simulink model "TestbedModel_v6"  (R2016a)
settings: Solver=ode23tb  StartTime=0.0  StopTime=20  RelTol=1e-3
undefined symbols (not defined in the file): K, Ki, Kp, magnitude, rev_comms_sink, tau
libraries: DAEMOT_Lib x4
(part 1 of 4)
settings Model: Creator=aksland2  LastModifiedBy=aksland2

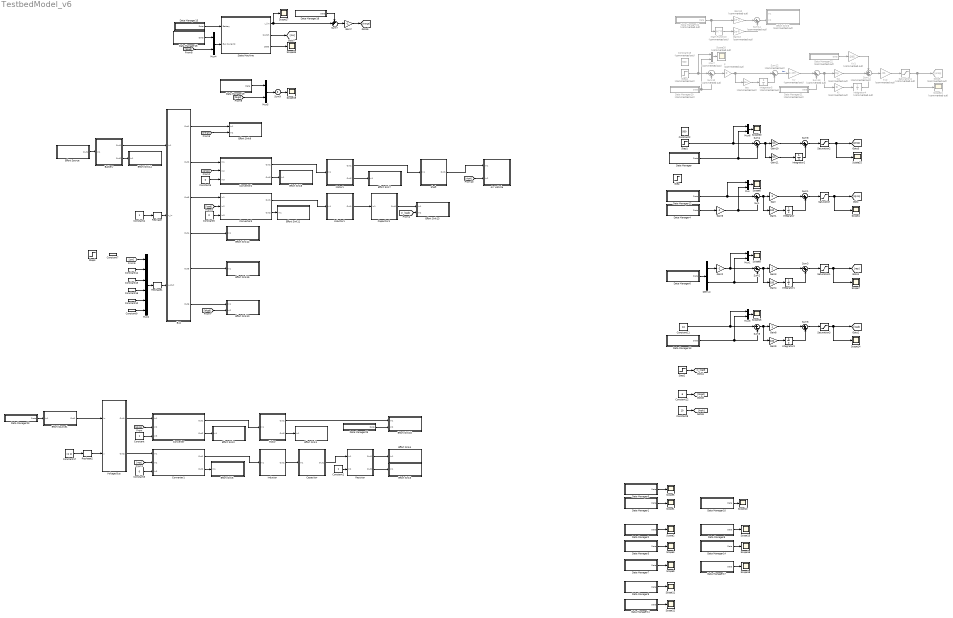
== system TestbedModel_v6 ==
  Air Vehicle : Subsystem  AncestorBlock=DAEMOT_Lib/Dyn Electrical Comp/Air Vehicle  mask{rho=1.225, g=9.81, M=69.5*.4536, A=2*pi*.3^2, C_D=1.5/45, v_initial=0, prop=AFRL}
      mask prompts: rho "Air Density [kg/m^3]"; g "Gravity [m/s^2]"; M "Vehicle Mass [kg]"; A "Frontal Area [m^2]"; C_D "Drag Coefficient [-]"; v_initial "Initial Vehicle Speed [m/s]"; prop "Propeller Map (filename)"
      mask init:
      | map = load('PropellerProp','PropellerProp');
      | Prop = eval(['map.PropellerProp.' prop]);
      | d = Prop.d;
      settings: CopyFcn=|
      | h      = get_param(gcb,'handle');   % Get block handle
      | blk    = gcb;
      | 
      | set_param(blk, 'LinkStatus', 'inactive')
      | clear h
      | clear blk
      mask Display:
      | image(imread('UAV.bmp'));
      | text(0.5,0.95,['{\bf UAV}'],'TexMode','on','horizontalAlignment', 'center')
      | text(0.5,0.075,['{\bf (\tau)  (end)}'],'TexMode','on','horizontalAlignment', 'center')
      | 
      | port_label('input',1,sprintf('Mechanical \nIn'))
      | % port_label('input',2,sprintf('\\lambda %g\t',10))
      | port_label('input',2,'\theta [rad]','interpreter','tex')
  Battery : Subsystem  AncestorBlock=DAEMOT_Lib/Dyn Electrical Comp/Battery  mask{C_c=62.7, C_s=4.5, R_cond=1.94, B_cap=21.33, Ns=1, Np=1, batt=57.6 Testbed 21.33 Ah, Ts_initial=25, Tc_initial=25, SOC_initial=.75, RC_initial=[0 0]}
      mask prompts: C_c "Lumped Cell Core Heat Capacity [J/K]"; C_s "Lumped Cell Surface Heat Capacity [J/K]"; R_cond "Conduction Resistance  [K/W]"; B_cap "Battery Capacity [Ah]"; Ns "Number of Cells (Series)"; Np "Number of Cells (Parallel)"; batt "Battery Type"; Ts_initial "Initial Battery Surface Temperature [C]"; Tc_initial "Initial Battery Core Temperature [C]"; SOC_initial "Initial State of Charge"; RC_initial "Initial RC Pair Voltage"
      mask init:
      | load('BattProp.mat');
      | 
      | if strcmp(batt,'3.3V LiFePO4 2.3 Ah')
      |     cell = BattProp.LiFePO_33V;
      |     t = 1;
      | end
      | 
      | if strcmp(batt,'3.3V LiFePO4 Graph 2.3 Ah')
      |     cell = BattProp.LiFePO_33V_G;
      |     t = 2;
      | end
      | 
      | if strcmp(batt,'4.2V LiPo 5.1 Ah')
      |     cell = BattProp.LiPo_42V;
      |     t = 1;
      | end
      | 
      | if strcmp(batt,'4.2V LiPo Graph 5.1 Ah')
      |     cell = BattProp.LiPo_42V_G;
      |     t = 2;
      | end
      | 
      | if strcmp(batt,'57.6 Testbed 21.33 Ah')
      |     cell = BattProp.Testbed4Pack;
      |     t = 1;
      | end
      | 
      | if strcmp(batt,'57.6 Testbed Graph 21.33 Ah')
      |     cell = BattProp.Testbed4Pack_G;
      |     t = 2;
      | end
      | 
      | 
      | % B_cap = B_cap*Np;
      | % C_c = C_c*Np*Ns;
      | % C_s = C_s*Np*Ns;
      | % R_cond = R_cond/(Np*Ns);
      settings: CopyFcn=|
      | h      = get_param(gcb,'handle');   % Get block handle
      | blk    = gcb;
      | 
      | set_param(blk, 'LinkStatus', 'inactive')
      | clear h
      | clear blk
      mask TypeOptions batt: 3.3V LiFePO4 2.3 Ah | 3.3V LiFePO4 Graph 2.3 Ah | 4.2V LiPo 5.1 Ah | 4.2V LiPo Graph 5.1 Ah | 57.6 Testbed 21.33 Ah | 57.6 Testbed Graph 21.33 Ah
      mask Display:
      | image(imread('battery.bmp'))
      | N = get_param(gcb,'Np');
      | M = get_param(gcb,'Ns');
      | 
      | text(0.5,0.95,[M '{\bfS}' N '{\bfP Battery}'],'TexMode','on','horizontalAlignment', 'center')
      | text(0.5,0.075,['{\bf (V)*}'],'TexMode','on','horizontalAlignment', 'center')
      | 
      | port_label('input',1,sprintf('Electrical \nIn'))
      | 
      | port_label('output',1,sprintf('Electrical \nOut'))
      | port_label('output',2,sprintf('Cooling \nOut'))
  Bus : Subsystem  AncestorBlock=DAEMOT_Lib/Dyn Electrical Comp/Bus  mask{R=5e-4, L=4e-8, C=.01, Num_In=1, Num_Out=6, V_initial=60, I_initial=0}
      mask prompts: R "Resistance [Ohm]"; L "Inductance [H]"; C "Capacitance [F]"; Num_In "Number of Inputs"; Num_Out "Number of Outputs"; V_initial "Initial Voltage [V]"; I_initial "Initial Current [A]"
      mask init:
      | h      = get_param(gcb,'handle');   % Get block handle
      | blk    = gcb;
      | hblock = get(h);     % Parse out handles structure
      | 
      | %%%%%%%%%%%%%%%%%%%%%%%%%%%%%% Clear Stuff %%%%%%%%%%%%%%%%%%%%%%%%%%%%%%%%
      | %delete any previous inports and bus selectors
      | for i = str2num(hblock.Num_In)+1:hblock.Ports(1)-2
      |     delete_block([blk,'/In',num2str(i)])
      |     delete_block([blk,'/gb',num2str(i)])
      |     delete_block([blk,'/vm',num2str(i)])
      |     delete_block([blk,'/term',num2str(i)])
      |     delete_block([blk,'/Sink',num2str(i)])
      |     delete_block([blk,'/vin',num2str(i)])
      |     
      |     delete_unconnected_lines(blk)
      | end
      | 
      | for i = str2num(hblock.Num_Out)+1:hblock.Ports(2)
      |     delete_block([blk,'/Out',num2str(i)])
      |     delete_block([blk,'/if',num2str(i)])
      |     delete_block([blk,'/io',num2str(i)])
      |     delete_block([blk,'/vo',num2str(i)])
      |     delete_block([blk,'/vot',num2str(i)])
      |     delete_block([blk,'/b',num2str(i)])
      |     delete_block([blk,'/Source',num2str(i)])
      |     delete_block([blk,'/ig',num2str(i)])
      | %     delete_block([blk,'/ios',num2str(i)])
      |     
      |     delete_unconnected_lines(blk)
      | end
      | %%%%%%%%%%%%%%%%%%%%%%%%%%%%% Clear Stuff %%%%%%%%%%%%%%%%%%%%%%%%%%%%%%%%
      | 
      | %%%%%%%%%%%%%%%%%%%%%%%%%%%%%% Edit Mux inputs %%%%%%%%%%%%%%%%%%%%%%%%%%%%%%%%
      | set_param([blk,'/Mux_In_1'],'Inputs',hblock.Num_In)
      | set_param([blk,'/Mux_In_2'],'Inputs',hblock.Num_Out)
      | set_param([blk,'/Demux_Out_1'],'Outputs',hblock.Num_In)
      | set_param([blk,'/Demux_Out_2'],'Outputs',hblock.Num_Out)
      | set_param([blk,'/u_Out'],'Port',num2str(Num_In+2))
      | set_param([blk,'/u_In'],'Port',num2str(Num_In+1))
      | set_param([blk,'/Bus_Sink_1'],'Inputs',num2str(str2num(hblock.Num_In)+1))
      | set_param([blk,'/Demux_Out_3'],'Outputs',hblock.Num_In)
      | delete_unconnected_lines(blk)
      | 
      | %%%%%%%%%%%%%%%%%%%%%%%%%%%%%% Edit Mux inputs %%%%%%%%%%%%%%%%%%%%%%%%%%%%%%%%
      | 
      | %%%%%%%%%%%%%%%%%%%%%%%%%%%%%% Create and Place Inputs %%%%%%%%%%%%%%%%%%%%%%%%%%%%%%%%
      | % generate inports, bus selectors, and route lines to each vector concat
      | for i = hblock.Ports(1)+1-2:str2num(hblock.Num_In)
      |     
      |     % add blocks (positioning notation [x i*s+y x+l i*s+h+y] x:(horiz. pos.), y:(vert. pos.), s:(spacing), l:(horiz. length), x:(vert. height)
      |     add_block('simulink/Ports & Subsystems/In1',   [blk,'/In',num2str(i)],    'Position',[355 i*80+425 355+30 i*80+13+425]);         % adding inport
      |     add_block([blk,'/gb1'],                        [blk,'/gb',num2str(i)],   'Position',[440 i*80+410 440+5 i*80+38+410]);         % adding inport
      |     add_block('simulink/Signal Routing/Goto',      [blk,'/vm',num2str(i)],    'Position',[500 i*80+450 500+80 i*80+14+450]);         % adding inport
      |     add_block('simulink/Sinks/Terminator',          [blk,'/term',num2str(i)],    'Position',[500 i*80+415 500+20 i*80+14+415]);         % adding inport
      |     add_block('DAEMOT_Lib/Support Functions/Sink',[blk,'/Sink',num2str(i)],'Position',[200 i*30+336 200+65 i*30+28+336]);         % adding inport
      |     add_block('simulink/Signal Routing/From',       [blk,'/vin',num2str(i)],     'Position',[-400 i*20+405 -400+80 i*20+18+405]);         % adding inport
      |     
      |     % set goto and from tags
      |     set_param([blk,'/vm',num2str(i)],'GotoTag',char(horzcat('V_in',num2str(i))))
      |     set_param([blk,'/vin',num2str(i)],'GotoTag',char(horzcat('V_in',num2str(i))))
      |     
      |     % set goto and from background colors
      | %    set_param([blk,'/gm',num2str(i)],'BackgroundColor','yellow')
      | %    set_param([blk,'/gt',num2str(i)],'BackgroundColor','yellow')
      | %    %set_param([blk,'/gp',num2str(i)],'BackgroundColor','yellow')
      | %    set_param([blk,'/min',num2str(i)],'BackgroundColor','yellow')
      | %    set_param([blk,'/tin',num2str(i)],'BackgroundColor','yellow')
      | %    set_param([blk,'/pout',num2str(i)],'BackgroundColor','cyan')
      |     
      |     % add lines
      |     add_line(blk,['In',num2str(i),'/1'], ['gb',num2str(i),'/1'],'AutoRouting','on')
      |     add_line(blk,['gb',num2str(i),'/2'],  ['vm',num2str(i),'/1'],'AutoRouting','on')
      |     add_line(blk,['gb',num2str(i),'/1'],  ['term',num2str(i),'/1'],'AutoRouting','on')
      |     add_line(blk,['Demux_Out_1/',num2str(i)],  ['Sink',num2str(i),'/1'],'AutoRouting','on')
      |     add_line(blk,['vin',num2str(i),'/1'],  ['Mux_In_1/',num2str(i)],'AutoRouting','on')
      |     add_line(blk,['Demux_Out_3/',num2str(i)'],  ['Bus_Sink_1/',num2str(i)+1],'AutoRouting','on')
      |     
      |     p = get_param([blk,'/Demux_Out_3'],'PortHandles');
      |     l = get_param(p.Outport(i),'Line');
      |     set_param(l,'Name',['Current',num2str(i),' [A]'])
      | %     
      | end
      | %%%%%%%%%%%%%%%%%%%%%%%%%%%%%% Create and Place Inputs %%%%%%%%%%%%%%%%%%%%%%%%%%%%%%%%
      | 
      | %%%%%%%%%%%%%%%%%%%%%%%%%%%%%% Create and Place Outputs %%%%%%%%%%%%%%%%%%%%%%%%%%%%%%%%
      | % generate inports, bus selectors, and route lines to each vector concat
      | for i = hblock.Ports(2)+1:str2num(hblock.Num_Out)
      |     
      |     % add blocks
      |     add_block('simulink/Ports & Subsystems/Out1',   [blk,'/Out',num2str(i)],   'Position',[875 i*80+425 875+30 i*80+13+425]);         % adding inport
      |     add_block('simulink/Signal Routing/Bus Creator',[blk,'/b',num2str(i)],     'Position',[825 i*80+410 825+5 i*80+38+410]);         % adding inport
      |     add_block('simulink/Signal Routing/From',       [blk,'/io',num2str(i)],     'Position',[710 i*80+415 710+80 i*80+14+415]);         % adding inport
      |     add_block('simulink/Signal Routing/From',       [blk,'/vo',num2str(i)],     'Position',[710 i*80+435 710+80 i*80+14+435]);         % adding inport
      |     add_block('simulink/Signal Routing/Goto',       [blk,'/vot',num2str(i)],     'Position',[1250 i*20+50 1250+80 i*20+18+50]);         % adding inport
      |     add_block('simulink/Signal Routing/From',       [blk,'/if',num2str(i)],     'Position',[935 i*20+410 935+80 i*20+18+410]);         % adding inport
      |     add_block('DAEMOT_Lib/Support Functions/Source',[blk,'/Source',num2str(i)],'Position',[1400 i*30+420 1400+65 i*30+28+420]);         % adding inport
      |     add_block('simulink/Signal Routing/Goto',       [blk,'/ig',num2str(i)],     'Position',[1550 i*30+430 1550+80 i*30+14+430]);         % adding inport
      | %     add_block('simulink/Signal Routing/From',       [blk,'/ios',num2str(i)],     'Position',[1770 i*16+405 1770+80 i*16+14+405]);         % adding inport
      |     
      |     % set goto and from tags
      |     set_param([blk,'/if',num2str(i)],'GotoTag',char(horzcat('I_out',num2str(i))))
      |     set_param([blk,'/io',num2str(i)],'GotoTag',char(horzcat('I_out',num2str(i))))
      |     set_param([blk,'/vo',num2str(i)],'GotoTag',char(horzcat('V_out',num2str(i))))
      |     set_param([blk,'/vot',num2str(i)],'GotoTag',char(horzcat('V_out',num2str(i))))
      |     set_param([blk,'/ig',num2str(i)],'GotoTag',char(horzcat('I_out',num2str(i))))
      | %     set_param([blk,'/ios',num2str(i)],'GotoTag',char(horzcat('I_out',num2str(i))))
      |     set_param([blk,'/b',num2str(i)],'Inputs','2')
      |     
      | %     % set goto and from background colors
      | %     set_param([blk,'/t',num2str(i)],'BackgroundColor','cyan')
      | %     set_param([blk,'/m',num2str(i)],'BackgroundColor','cyan')
      | %     set_param([blk,'/p',num2str(i)],'BackgroundColor','cyan')
      | %     set_param([blk,'/g',num2str(i)],'BackgroundColor','cyan')
      | %     set_param([blk,'/mout',num2str(i)],'BackgroundColor','cyan')
      | %     %set_param([blk,'/tout',num2str(i)],'BackgroundColor','cyan')
      |     
      |     % add lines
      |     add_line(blk,['io',num2str(i),'/1'],['b',num2str(i),'/1'],'AutoRouting','on')
      |     p = get_param([blk,'/io',num2str(i)],'PortHandles');
      |     l = get_param(p.Outport,'Line');
      |     set_param(l,'Name','current')
      |     
      |     add_line(blk,['vo',num2str(i),'/1'],['b',num2str(i),'/2'],'AutoRouting','on')
      |     p = get_param([blk,'/vo',num2str(i)],'PortHandles');
      |     l = get_param(p.Outport,'Line');
      |     set_param(l,'Name','voltage')
      |         
      | %     add_line(blk,['ios',num2str(i),'/1'],['Bus_Sink_1/',num2str(i+1)],'AutoRouting','on')
      | %     p = get_param([blk,'/ios',num2str(i)],'PortHandles');
      | %     l = get_param(p.Outport,'Line');
      | %     set_param(l,'Name',['Current',num2str(i),' [A]'])
      |      
      |     add_line(blk,['b',num2str(i),'/1'],['Out',num2str(i),'/1'],'AutoRouting','on')
      |     add_line(blk,['Source',num2str(i),'/1'],['ig',num2str(i),'/1'],'AutoRouting','on')
      |     add_line(blk,['if',num2str(i),'/1'],  ['Mux_In_2/',num2str(i)],'AutoRouting','on')
      |     add_line(blk,['Demux_Out_2/',num2str(i)],['vot',num2str(i),'/1'],'AutoRouting','on')
      |     
      | 
      | 
      | end
      | %%%%%%%%%%%%%%%%%%%%%%%%%%%%%% Create and Place Outputs %%%%%%%%%%%%%%%%%%%%%%%%%%%%%%%%
      | 
      | try
      |     set_param([blk,'/Selector1'],'InputPortWidth',num2str(hblock.Num_In))
      |     
      |     selector_str = '[1 ';
      |     for i = 2:str2num(hblock.Num_In)
      |         selector_str = [selector_str,num2str(i),' '];
      |     end
      |     selector_str = [selector_str,']'];
      |     set_param([blk,'/Selector1'],'IndexParamArray',{selector_str})%num2cell(1:hblock.Num_In))
      | catch
      |     selector_str = '[1 ';
      |     for i = 2:str2num(hblock.Num_In)
      |         selector_str = [selector_str,num2str(i),' '];
      |     end
      |     selector_str = [selector_str,']'];
      |     set_param([blk,'/Selector1'],'IndexParamArray',{selector_str})%num2cell(1:hblock.Num_In))
      |     
      |     set_param([blk,'/Selector1'],'InputPortWidth',num2str(hblock.Num_In))
      | end 
      |     
      | try
      |     set_param([blk,'/Selector2'],'InputPortWidth',num2str(hblock.Num_Out))
      |     
      |     selector_str = '[1 ';
      |     for i = 2:str2num(hblock.Num_Out)
      |         selector_str = [selector_str,num2str(i),' '];
      |     end
      |     selector_str = [selector_str,']'];
      |     set_param([blk,'/Selector2'],'IndexParamArray',{selector_str})%num2cell(1:hblock.Num_Out))
      | catch
      |     selector_str = '[1 ';
      |     for i = 2:str2num(hblock.Num_Out)
      |         selector_str = [selector_str,num2str(i),' '];
      |     end
      |     selector_str = [selector_str,']'];
      |     set_param([blk,'/Selector2'],'IndexParamArray',{selector_str})%num2cell(1:hblock.Num_Out))
      |     
      |     set_param([blk,'/Selector2'],'InputPortWidth',num2str(hblock.Num_Out))
      | end 
      | 
      |     clear h blk hblock
      settings: CopyFcn=|
      | h      = get_param(gcb,'handle');   % Get block handle
      | blk    = gcb;
      | 
      | set_param(blk, 'LinkStatus', 'inactive')
      | clear h
      | clear blk
      mask Display:
      | text(0.5,0.95,['{\bf Bus}'],'TexMode','on','horizontalAlignment', 'center')
      | text(0.5,0.075,['{\bf ----(V)}'],'TexMode','on','horizontalAlignment', 'center')
      | 
      | In = get_param(gcb,'Num_In');
      | Out = get_param(gcb,'Num_Out');
      | 
      | for i = 1:str2num(In)
      |     port_label('input',i,sprintf(['Electrical \nIn ',num2str(i)]))
      | end
      | port_label('input',str2num(In)+1,'u In')
      | port_label('input',str2num(In)+2,'u Out')
      | 
      | for i = 1:str2num(Out)
      |     port_label('output',i,sprintf(['Electrical \nOut ',num2str(i)]))
      | end
  Capacitor : Subsystem  AncestorBlock=DAEMOT_Lib/Dyn Electrical Comp/Capacitor  mask{C=.003, V_initial=0}
      mask prompts: C "Capacitance [F]"; V_initial "Initial Ouput Voltage [V]"
      mask init:
      | % if strcmp(Gn_check,'off')
      | %     %is not ground node
      | %     Gn = 0;
      | %     %V_initial = V_initial_temp;
      | % else
      | %     %is ground node
      | %     Gn = 1;
      | %     %V_initial = 0;
      | % end
      settings: CopyFcn=|
      | h      = get_param(gcb,'handle');   % Get block handle
      | blk    = gcb;
      | 
      | set_param(blk, 'LinkStatus', 'inactive')
      | clear h
      | clear blk
      mask Display:
      | image(imread('capacitor.bmp'));
      | text(0.5,0.95,['{\bf Capacitor}'],'TexMode','on','horizontalAlignment', 'center')
      | text(0.5,0.075,['{\bf (V)}'],'TexMode','on','horizontalAlignment', 'center')
      | 
      | port_label('input',1,sprintf('Electrical \nIn'))
      | %port_label('input',2,'Capacitance')
      | port_label('output',1,sprintf('Electrical \nOut'))
  Capacitor1 : Subsystem  AncestorBlock=DAEMOT_Lib/Dyn Electrical Comp/Capacitor  mask{C=.003, V_initial=24}
      mask prompts: C "Capacitance [F]"; V_initial "Initial Ouput Voltage [V]"
      mask init:
      | % if strcmp(Gn_check,'off')
      | %     %is not ground node
      | %     Gn = 0;
      | %     %V_initial = V_initial_temp;
      | % else
      | %     %is ground node
      | %     Gn = 1;
      | %     %V_initial = 0;
      | % end
      settings: CopyFcn=|
      | h      = get_param(gcb,'handle');   % Get block handle
      | blk    = gcb;
      | 
      | set_param(blk, 'LinkStatus', 'inactive')
      | clear h
      | clear blk
      mask Display:
      | image(imread('capacitor.bmp'));
      | text(0.5,0.95,['{\bf Capacitor}'],'TexMode','on','horizontalAlignment', 'center')
      | text(0.5,0.075,['{\bf (V)}'],'TexMode','on','horizontalAlignment', 'center')
      | 
      | port_label('input',1,sprintf('Electrical \nIn'))
      | %port_label('input',2,'Capacitance')
      | port_label('output',1,sprintf('Electrical \nOut'))
  Constant{,1,4,9..10,14..16} (8 alike) : Constant
  Constant11 : Constant  Value=24
  Constant12 : Constant  Value=.5
  Constant13 : Constant  Commented=on  Value=500
  Constant17 : Constant  Value=[1 1]
  Constant2 : Constant  Value=500
  Constant{3,5..7} (4 alike) : Constant  Value=0
  Constant8 : Constant  Value=10
  Converter : Subsystem  AncestorBlock=DAEMOT_Lib/Dyn Electrical Comp/Converter  mask{V_D=.01, R_D=.01, R_s=.01, R_L=.01, dir=<===, Cp=60, T_initial=25}
      mask prompts: V_D "Diode Voltage Difference [V]"; R_D "Diode Resistance [Ohm]"; R_s "Switch Resistance [Ohm]"; R_L "Copper Loss [Ohm]"; dir "Conversion Direction (Boost)"; Cp "Heat Capacity [J/K]"; T_initial "Initial Temperature [C]"
      settings: CopyFcn=|
      | h      = get_param(gcb,'handle');   % Get block handle
      | blk    = gcb;
      | 
      | set_param(blk, 'LinkStatus', 'inactive')
      | clear h
      | clear blk
      mask TypeOptions dir: ===> | <===
      mask Display:
      | image(imread('converter.bmp'));
      | text(0.5,0.95,['{\bf BuckBoost Converter}'],'TexMode','on','horizontalAlignment', 'center')
      | text(0.5,0.075,['{\bf ----(V)}'],'TexMode','on','horizontalAlignment', 'center')
      | dir = get_param(gcb,'dir');
      | 
      | switch dir
      |     case '===>'
      |         text(0.5,0.85,['{\bf Boost[1] ===>}'],'TexMode','on','horizontalAlignment', 'center')
      |         text(0.5,0.75,['{\bf Buck[0] <===}'],'TexMode','on','horizontalAlignment', 'center')
      |     case '<==='
      |         text(0.5,0.85,['{\bf Boost[1] <===}'],'TexMode','on','horizontalAlignment', 'center')
      |         text(0.5,0.75,['{\bf Buck[0] ===>}'],'TexMode','on','horizontalAlignment', 'center')
      | end
      | 
      | 
      | 
      | port_label('input',1,sprintf('Electrical \nIn'))
      | port_label('input',2,sprintf('Duty \nCycle'))
      | port_label('input',3,sprintf('Operating \nMode'))
      | port_label('output',1,sprintf('Electrical \nOut'))
      | port_label('output',2,sprintf('Cooling \nOut'))
  Converter1 : Subsystem  AncestorBlock=DAEMOT_Lib/Dyn Electrical Comp/Converter  mask{V_D=.01, R_D=.01, R_s=.01, R_L=.01, dir=<===, Cp=60, T_initial=25}
      mask prompts: V_D "Diode Voltage Difference [V]"; R_D "Diode Resistance [Ohm]"; R_s "Switch Resistance [Ohm]"; R_L "Copper Loss [Ohm]"; dir "Conversion Direction (Boost)"; Cp "Heat Capacity [J/K]"; T_initial "Initial Temperature [C]"
      settings: CopyFcn=|
      | h      = get_param(gcb,'handle');   % Get block handle
      | blk    = gcb;
      | 
      | set_param(blk, 'LinkStatus', 'inactive')
      | clear h
      | clear blk
      mask TypeOptions dir: ===> | <===
      mask Display:
      | image(imread('converter.bmp'));
      | text(0.5,0.95,['{\bf BuckBoost Converter}'],'TexMode','on','horizontalAlignment', 'center')
      | text(0.5,0.075,['{\bf ----(V)}'],'TexMode','on','horizontalAlignment', 'center')
      | dir = get_param(gcb,'dir');
      | 
      | switch dir
      |     case '===>'
      |         text(0.5,0.85,['{\bf Boost[1] ===>}'],'TexMode','on','horizontalAlignment', 'center')
      |         text(0.5,0.75,['{\bf Buck[0] <===}'],'TexMode','on','horizontalAlignment', 'center')
      |     case '<==='
      |         text(0.5,0.85,['{\bf Boost[1] <===}'],'TexMode','on','horizontalAlignment', 'center')
      |         text(0.5,0.75,['{\bf Buck[0] ===>}'],'TexMode','on','horizontalAlignment', 'center')
      | end
      | 
      | 
      | 
      | port_label('input',1,sprintf('Electrical \nIn'))
      | port_label('input',2,sprintf('Duty \nCycle'))
      | port_label('input',3,sprintf('Operating \nMode'))
      | port_label('output',1,sprintf('Electrical \nOut'))
      | port_label('output',2,sprintf('Cooling \nOut'))
  Converter2 : Subsystem  AncestorBlock=DAEMOT_Lib/Dyn Electrical Comp/Converter  mask{V_D=.05, R_D=.01, R_s=.01, R_L=.01, dir=<===, Cp=60, T_initial=25}
      mask prompts: V_D "Diode Voltage Difference [V]"; R_D "Diode Resistance [Ohm]"; R_s "Switch Resistance [Ohm]"; R_L "Copper Loss [Ohm]"; dir "Conversion Direction (Boost)"; Cp "Heat Capacity [J/K]"; T_initial "Initial Temperature [C]"
      settings: CopyFcn=|
      | h      = get_param(gcb,'handle');   % Get block handle
      | blk    = gcb;
      | 
      | set_param(blk, 'LinkStatus', 'inactive')
      | clear h
      | clear blk
      mask TypeOptions dir: ===> | <===
      mask Display:
      | image(imread('converter.bmp'));
      | text(0.5,0.95,['{\bf BuckBoost Converter}'],'TexMode','on','horizontalAlignment', 'center')
      | text(0.5,0.075,['{\bf ----(V)}'],'TexMode','on','horizontalAlignment', 'center')
      | dir = get_param(gcb,'dir');
      | 
      | switch dir
      |     case '===>'
      |         text(0.5,0.85,['{\bf Boost[1] ===>}'],'TexMode','on','horizontalAlignment', 'center')
      |         text(0.5,0.75,['{\bf Buck[0] <===}'],'TexMode','on','horizontalAlignment', 'center')
      |     case '<==='
      |         text(0.5,0.85,['{\bf Boost[1] <===}'],'TexMode','on','horizontalAlignment', 'center')
      |         text(0.5,0.75,['{\bf Buck[0] ===>}'],'TexMode','on','horizontalAlignment', 'center')
      | end
      | 
      | 
      | 
      | port_label('input',1,sprintf('Electrical \nIn'))
      | port_label('input',2,sprintf('Duty \nCycle'))
      | port_label('input',3,sprintf('Operating \nMode'))
      | port_label('output',1,sprintf('Electrical \nOut'))
      | port_label('output',2,sprintf('Cooling \nOut'))
  Converter3 : Subsystem  AncestorBlock=DAEMOT_Lib/Dyn Electrical Comp/Converter  mask{V_D=.05, R_D=.01, R_s=.01, R_L=.01, dir=<===, Cp=60, T_initial=25}
      mask prompts: V_D "Diode Voltage Difference [V]"; R_D "Diode Resistance [Ohm]"; R_s "Switch Resistance [Ohm]"; R_L "Copper Loss [Ohm]"; dir "Conversion Direction (Boost)"; Cp "Heat Capacity [J/K]"; T_initial "Initial Temperature [C]"
      settings: CopyFcn=|
      | h      = get_param(gcb,'handle');   % Get block handle
      | blk    = gcb;
      | 
      | set_param(blk, 'LinkStatus', 'inactive')
      | clear h
      | clear blk
      mask TypeOptions dir: ===> | <===
      mask Display:
      | image(imread('converter.bmp'));
      | text(0.5,0.95,['{\bf BuckBoost Converter}'],'TexMode','on','horizontalAlignment', 'center')
      | text(0.5,0.075,['{\bf ----(V)}'],'TexMode','on','horizontalAlignment', 'center')
      | dir = get_param(gcb,'dir');
      | 
      | switch dir
      |     case '===>'
      |         text(0.5,0.85,['{\bf Boost[1] ===>}'],'TexMode','on','horizontalAlignment', 'center')
      |         text(0.5,0.75,['{\bf Buck[0] <===}'],'TexMode','on','horizontalAlignment', 'center')
      |     case '<==='
      |         text(0.5,0.85,['{\bf Boost[1] <===}'],'TexMode','on','horizontalAlignment', 'center')
      |         text(0.5,0.75,['{\bf Buck[0] ===>}'],'TexMode','on','horizontalAlignment', 'center')
      | end
      | 
      | 
      | 
      | port_label('input',1,sprintf('Electrical \nIn'))
      | port_label('input',2,sprintf('Duty \nCycle'))
      | port_label('input',3,sprintf('Operating \nMode'))
      | port_label('output',1,sprintf('Electrical \nOut'))
      | port_label('output',2,sprintf('Cooling \nOut'))
  Data Manager : Subsystem  AncestorBlock=DAEMOT_Lib/Support Functions/Data Manager  mask{null=0}
      mask init:
      | set_param(gcb, 'LinkStatus', 'inactive')    % disable the library link
      settings: OpenFcn=data_manager
      mask Display: str ='Shaft/Speed [rad_s]'; fprintf(str)
  Data Manager1 : Subsystem  AncestorBlock=DAEMOT_Lib/Support Functions/Data Manager  mask{null=0}
      mask init:
      | set_param(gcb, 'LinkStatus', 'inactive')    % disable the library link
      settings: OpenFcn=data_manager
      mask Display: str ='Converter/Current In [A]'; fprintf(str)
  Data Manager10 : Subsystem  AncestorBlock=DAEMOT_Lib/Support Functions/Data Manager  mask{null=0}
      mask init:
      | set_param(gcb, 'LinkStatus', 'inactive')    % disable the library link
      settings: OpenFcn=data_manager
      mask Display: str ='Converter1/Current In [A]'; fprintf(str)
  Data Manager11 : Subsystem  AncestorBlock=DAEMOT_Lib/Support Functions/Data Manager  mask{null=0}
      mask init:
      | set_param(gcb, 'LinkStatus', 'inactive')    % disable the library link
      settings: OpenFcn=data_manager
      mask Display: str ='Motor1/Torque [Nm]'; fprintf(str)
  Data Manager12 : Subsystem  AncestorBlock=DAEMOT_Lib/Support Functions/Data Manager  mask{null=0}
      mask init:
      | set_param(gcb, 'LinkStatus', 'inactive')    % disable the library link
      settings: OpenFcn=data_manager
      mask Display: str ='Air Vehicle/Load Torque [Nm]'; fprintf(str)
  Data Manager13 : Subsystem  AncestorBlock=DAEMOT_Lib/Support Functions/Data Manager  mask{null=0}
      mask init:
      | set_param(gcb, 'LinkStatus', 'inactive')    % disable the library link
      settings: OpenFcn=data_manager
      mask Display: str ='Capacitor1/Voltage [V]'; fprintf(str)
  Data Manager14 : Subsystem  AncestorBlock=DAEMOT_Lib/Support Functions/Data Manager  mask{null=0}
      mask init:
      | set_param(gcb, 'LinkStatus', 'inactive')    % disable the library link
      settings: OpenFcn=data_manager
      mask Display: str ='Battery/SOC [-]'; fprintf(str)
  Data Manager15 : Subsystem  AncestorBlock=DAEMOT_Lib/Support Functions/Data Manager  mask{null=0}
      mask init:
      | set_param(gcb, 'LinkStatus', 'inactive')    % disable the library link
      settings: OpenFcn=data_manager
      mask Display: str ='Battery/SOC [-]\nBattery/Current [A]'; fprintf(str)
  Data Manager16 : Subsystem  AncestorBlock=DAEMOT_Lib/Support Functions/Data Manager  mask{null=0}
      mask init:
      | set_param(gcb, 'LinkStatus', 'inactive')    % disable the library link
      settings: OpenFcn=data_manager
      mask Display: str ='Converter2/Current In [A]\nConverter/Current In [A]\nConverter1/Current In [A]\nConverter3/Current In [A]'; fprintf(str)
  Data Manager17 : Subsystem  AncestorBlock=DAEMOT_Lib/Support Functions/Data Manager  mask{null=0}
      mask init:
      | set_param(gcb, 'LinkStatus', 'inactive')    % disable the library link
      settings: OpenFcn=data_manager
      mask Display: str ='Battery/Current [A]'; fprintf(str)
  Data Manager18 : Subsystem  AncestorBlock=DAEMOT_Lib/Support Functions/Data Manager  mask{null=0}
      mask init:
      | set_param(gcb, 'LinkStatus', 'inactive')    % disable the library link
      settings: OpenFcn=data_manager
      mask Display: str ='Converter2/Current In [A]'; fprintf(str)
  Data Manager19 : Subsystem  AncestorBlock=DAEMOT_Lib/Support Functions/Data Manager  mask{null=0}
      mask init:
      | set_param(gcb, 'LinkStatus', 'inactive')    % disable the library link
      settings: OpenFcn=data_manager
      mask Display: str ='Converter2/Current In [A]\nConverter3/Current In [A]'; fprintf(str)
  Data Manager2 : Subsystem  AncestorBlock=DAEMOT_Lib/Support Functions/Data Manager  mask{null=0}
      mask init:
      | set_param(gcb, 'LinkStatus', 'inactive')    % disable the library link
      settings: OpenFcn=data_manager
      mask Display: str ='Motor/Current [A]'; fprintf(str)
  Data Manager20 : Subsystem  Commented=on  AncestorBlock=DAEMOT_Lib/Support Functions/Data Manager  mask{null=0}
      mask init:
      | set_param(gcb, 'LinkStatus', 'inactive')    % disable the library link
      settings: OpenFcn=data_manager
      mask Display: str ='Shaft/Speed [rad_s]'; fprintf(str)
  Data Manager21 : Subsystem  Commented=on  AncestorBlock=DAEMOT_Lib/Support Functions/Data Manager  mask{null=0}
      mask init:
      | set_param(gcb, 'LinkStatus', 'inactive')    % disable the library link
      settings: OpenFcn=data_manager
      mask Display: str ='Motor1/Current [A]'; fprintf(str)
  Data Manager22 : Subsystem  Commented=on  AncestorBlock=DAEMOT_Lib/Support Functions/Data Manager  mask{null=0}
      mask init:
      | set_param(gcb, 'LinkStatus', 'inactive')    % disable the library link
      settings: OpenFcn=data_manager
      mask Display: str ='Shaft/Speed [rad_s]'; fprintf(str)
  Data Manager23 : Subsystem  AncestorBlock=DAEMOT_Lib/Support Functions/Data Manager  mask{null=0}
      mask init:
      | set_param(gcb, 'LinkStatus', 'inactive')    % disable the library link
      settings: OpenFcn=data_manager
      mask Display: str ='Bus/Voltage [V]'; fprintf(str)
  Data Manager24 : Subsystem  Commented=on  AncestorBlock=DAEMOT_Lib/Support Functions/Data Manager  mask{null=0}
      mask init:
      | set_param(gcb, 'LinkStatus', 'inactive')    % disable the library link
      settings: OpenFcn=data_manager
      mask Display: str ='Shaft/Speed [rad_s]'; fprintf(str)
  Data Manager25 : Subsystem  AncestorBlock=DAEMOT_Lib/Support Functions/Data Manager  mask{null=0}
      mask init:
      | set_param(gcb, 'LinkStatus', 'inactive')    % disable the library link
      settings: OpenFcn=data_manager
      mask Display: str ='Shaft/Speed [rad_s]'; fprintf(str)
  Data Manager3 : Subsystem  AncestorBlock=DAEMOT_Lib/Support Functions/Data Manager  mask{null=0}
      mask init:
      | set_param(gcb, 'LinkStatus', 'inactive')    % disable the library link
      settings: OpenFcn=data_manager
      mask Display: str ='Converter/Voltage Out [V]'; fprintf(str)
  Data Manager4 : Subsystem  AncestorBlock=DAEMOT_Lib/Support Functions/Data Manager  mask{null=0}
      mask init:
      | set_param(gcb, 'LinkStatus', 'inactive')    % disable the library link
      settings: OpenFcn=data_manager
      mask Display: str ='Motor/Torque [Nm]'; fprintf(str)
  Data Manager5 : Subsystem  AncestorBlock=DAEMOT_Lib/Support Functions/Data Manager  mask{null=0}
      mask init:
      | set_param(gcb, 'LinkStatus', 'inactive')    % disable the library link
      settings: OpenFcn=data_manager
      mask Display: str ='Motor/Torque [Nm]'; fprintf(str)
  Data Manager6 : Subsystem  AncestorBlock=DAEMOT_Lib/Support Functions/Data Manager  mask{null=0}
      mask init:
      | set_param(gcb, 'LinkStatus', 'inactive')    % disable the library link
      settings: OpenFcn=data_manager
      mask Display: str ='Converter/Current In [A]\nConverter1/Current In [A]'; fprintf(str)
  Data Manager7 : Subsystem  AncestorBlock=DAEMOT_Lib/Support Functions/Data Manager  mask{null=0}
      mask init:
      | set_param(gcb, 'LinkStatus', 'inactive')    % disable the library link
      settings: OpenFcn=data_manager
      mask Display: str ='Bus/Current1 [A]'; fprintf(str)
  Data Manager8 : Subsystem  AncestorBlock=DAEMOT_Lib/Support Functions/Data Manager  mask{null=0}
      mask init:
      | set_param(gcb, 'LinkStatus', 'inactive')    % disable the library link
      settings: OpenFcn=data_manager
      mask Display: str ='Bus/Voltage [V]'; fprintf(str)
  Data Manager9 : Subsystem  AncestorBlock=DAEMOT_Lib/Support Functions/Data Manager  mask{null=0}
      mask init:
      | set_param(gcb, 'LinkStatus', 'inactive')    % disable the library link
      settings: OpenFcn=data_manager
      mask Display: str ='Motor1/Current [A]'; fprintf(str)
  Demux : Demux  Outputs=2
  Effort Sink1 : Subsystem  AncestorBlock=DAEMOT_Lib/Dyn Electrical Comp/Effort Sink  mask(Effort Sink (Torque)){Stype=Heat Flow Sink, const=on, value=1}
      mask prompts: Stype "Sink Type"; const "Constant Value?"; value "Heat Flow [kW]"
      mask help: Used to create a effot sink.
      mask init:
      | h      = get_param(gcb,'handle');   % Get block handle
      | blk    = gcb;
      | hblock = get(h);     % Parse out handles structure
      | 
      | if const == 1;
      |     try delete_block([blk,'/In2'])
      |         delete_unconnected_lines(blk);
      |         add_block('simulink/Sources/Constant',   [blk,'/val'], 'Position', [200,218,230,232]);
      |         add_line(blk,'val/1','Sink1/1','AutoRouting','on');
      |         set_param([blk,'/val'],'Value','value');
      |     end
      |      
      | %     delete_unconnected_lines(blk)
      | else
      |     try delete_block([blk,'/val'])
      |         delete_unconnected_lines(blk);
      |         add_block('simulink/Ports & Subsystems/In1',   [blk,'/In2'], 'Position', [200,218,230,232]);
      |         add_line(blk,'In2/1','Sink1/1','AutoRouting','on');
      |     end
      | end
      | 
      | clear h blk hblock
      settings: CopyFcn=|
      | h      = get_param(gcb,'handle');   % Get block handle
      | blk    = gcb;
      | 
      | set_param(blk, 'LinkStatus', 'inactive')
      | clear h
      | clear blk
      mask TypeOptions Stype: Voltage Sink | Current Sink | Angular Speed Sink | Torque Sink | Temperature Sink | Heat Flow Sink
      mask Callback Stype:
      | mp = get_param(gcb,'MaskPrompts');
      | h      = get_param(gcb,'handle');   % Get block handle
      | blk    = gcb;
      | hblock = get(h);     % Parse out handles structure
      | 
      | switch get_param(gcb,'Stype')
      |     case 'Voltage Sink'
      |         mp{3} = 'Voltage [V]';
      |     case 'Current Sink'
      |         mp{3} = 'Current [A]';
      |     case 'Angular Speed Sink'
      |         mp{3} = 'Speed [rad/s]';
      |     case 'Torque Sink'
      |         mp{3} = 'Torque [Nm]';
      |     case 'Temperature Sink'
      |         mp{3} = 'Temperature [C]';
      |     case 'Heat Flow Sink'
      |         mp{3} = 'Heat Flow [kW]';
      | end
      | set_param(gcb,'MaskPrompts',mp);
      mask Callback const:
      | en = get_param(gcb,'MaskVisibilities');
      | h      = get_param(gcb,'handle');   % Get block handle
      | blk    = gcb;
      | hblock = get(h);     % Parse out handles structure
      | 
      | switch get_param(gcb,'const')
      |     case 'on'
      |         en{3} = 'on';
      | %         delete_block([blk,'/In1'])
      | 
      |     case 'off'
      |         en{3} = 'off';
      | %         add_block('simulink/Ports & Subsystems/In1',   [blk,'/In1'],'Position',[130    -7   160     7]);         % adding inport
      | 
      | end
      | set_param(gcb,'MaskVisibilities',en);
      | 
      | % hblock.MaskPrompts{3} = 'hello';
      mask Display:
      | text(0.45,0.90,['{\bf',get_param(gcb,'Stype'),'}'],'TexMode','on','horizontalAlignment', 'center')
      | % text(0.5,0.1,['{(T)(end)}'],'TexMode','on','horizontalAlignment', 'center')
      | 
      | type = get_param(gcb,'Stype');
      | switch type
      |         case 'Voltage Sink'
      |             nm = 'Voltage [V]';
      |             id = '(V)';
      |             un = 'V';
      |         case 'Current Sink'
      |             nm = 'Current [A]';
      |             id = '(----)';
      |             un = 'A';
      |         case 'Angular Speed Sink'
      |             nm = 'Speed [rad/s]';
      |             id = '(----)';
      |             un = 'rad/s';
      |         case 'Torque Sink'
      |             nm = 'Torque [Nm]';
      |             id = '(\tau)';
      |             un = 'Nm';
      |         case 'Temperature Sink'
      |             nm = 'Temperature [C]';
      |             id = '(T)';
      |             un = 'C';
      |         case 'Heat Flow Sink'
      |             nm = 'Heat Flow [kW]';
      |             id = '(----)';
      |             un = 'kW';
      | end
      | 
      | if strcmp(get_param(gcb,'const'),'on')
      |     text(0.75,0.500,['{\bf',get_param(gcb,'Value'),un,'}'],'TexMode','on','horizontalAlignment', 'center')
      | else
      |     port_label('input',2,sprintf(['Sink ',nm]));
      | end
      | 
      | 
      | port_label('input',1,'Sink');
      | text(0.5,0.175,['{',id,' (end)}'],'TexMode','on','horizontalAlignment', 'center');
  Effort Sink10 : Subsystem  AncestorBlock=DAEMOT_Lib/Dyn Electrical Comp/Effort Sink  mask(Effort Sink (Torque)){Stype=Current Sink, const=off, value=.5}
      mask prompts: Stype "Sink Type"; const "Constant Value?"; value "Current [A]"
      mask help: Used to create a effot sink.
      mask init: same as TestbedModel_v6/Effort Sink1
      settings: CopyFcn=|
      | h      = get_param(gcb,'handle');   % Get block handle
      | blk    = gcb;
      | 
      | set_param(blk, 'LinkStatus', 'inactive')
      | clear h
      | clear blk
      mask TypeOptions Stype: Voltage Sink | Current Sink | Angular Speed Sink | Torque Sink | Temperature Sink | Heat Flow Sink
      mask Callback Stype:
      | mp = get_param(gcb,'MaskPrompts');
      | h      = get_param(gcb,'handle');   % Get block handle
      | blk    = gcb;
      | hblock = get(h);     % Parse out handles structure
      | 
      | switch get_param(gcb,'Stype')
      |     case 'Voltage Sink'
      |         mp{3} = 'Voltage [V]';
      |     case 'Current Sink'
      |         mp{3} = 'Current [A]';
      |     case 'Angular Speed Sink'
      |         mp{3} = 'Speed [rad/s]';
      |     case 'Torque Sink'
      |         mp{3} = 'Torque [Nm]';
      |     case 'Temperature Sink'
      |         mp{3} = 'Temperature [C]';
      |     case 'Heat Flow Sink'
      |         mp{3} = 'Heat Flow [kW]';
      | end
      | set_param(gcb,'MaskPrompts',mp);
      mask Callback const:
      | en = get_param(gcb,'MaskVisibilities');
      | h      = get_param(gcb,'handle');   % Get block handle
      | blk    = gcb;
      | hblock = get(h);     % Parse out handles structure
      | 
      | switch get_param(gcb,'const')
      |     case 'on'
      |         en{3} = 'on';
      | %         delete_block([blk,'/In1'])
      | 
      |     case 'off'
      |         en{3} = 'off';
      | %         add_block('simulink/Ports & Subsystems/In1',   [blk,'/In1'],'Position',[130    -7   160     7]);         % adding inport
      | 
      | end
      | set_param(gcb,'MaskVisibilities',en);
      | 
      | % hblock.MaskPrompts{3} = 'hello';
      mask Display:
      | text(0.45,0.90,['{\bf',get_param(gcb,'Stype'),'}'],'TexMode','on','horizontalAlignment', 'center')
      | % text(0.5,0.1,['{(T)(end)}'],'TexMode','on','horizontalAlignment', 'center')
      | 
      | type = get_param(gcb,'Stype');
      | switch type
      |         case 'Voltage Sink'
      |             nm = 'Voltage [V]';
      |             id = '(V)';
      |             un = 'V';
      |         case 'Current Sink'
      |             nm = 'Current [A]';
      |             id = '(----)';
      |             un = 'A';
      |         case 'Angular Speed Sink'
      |             nm = 'Speed [rad/s]';
      |             id = '(----)';
      |             un = 'rad/s';
      |         case 'Torque Sink'
      |             nm = 'Torque [Nm]';
      |             id = '(\tau)';
      |             un = 'Nm';
      |         case 'Temperature Sink'
      |             nm = 'Temperature [C]';
      |             id = '(T)';
      |             un = 'C';
      |         case 'Heat Flow Sink'
      |             nm = 'Heat Flow [kW]';
      |             id = '(----)';
      |             un = 'kW';
      | end
      | 
      | if strcmp(get_param(gcb,'const'),'on')
      |     text(0.75,0.500,['{\bf',get_param(gcb,'Value'),un,'}'],'TexMode','on','horizontalAlignment', 'center')
      | else
      |     port_label('input',2,sprintf(['Sink ',nm]));
      | end
      | 
      | 
      | port_label('input',1,'Sink');
      | text(0.5,0.175,['{',id,' (end)}'],'TexMode','on','horizontalAlignment', 'center');
  Effort Sink11 : Subsystem  AncestorBlock=DAEMOT_Lib/Dyn Electrical Comp/Effort Sink  mask(Effort Sink (Torque)){Stype=Heat Flow Sink, const=on, value=1}
      mask prompts: Stype "Sink Type"; const "Constant Value?"; value "Heat Flow [kW]"
      mask help: Used to create a effot sink.
      mask init: same as TestbedModel_v6/Effort Sink1
      settings: CopyFcn=|
      | h      = get_param(gcb,'handle');   % Get block handle
      | blk    = gcb;
      | 
      | set_param(blk, 'LinkStatus', 'inactive')
      | clear h
      | clear blk
      mask TypeOptions Stype: Voltage Sink | Current Sink | Angular Speed Sink | Torque Sink | Temperature Sink | Heat Flow Sink
      mask Callback Stype:
      | mp = get_param(gcb,'MaskPrompts');
      | h      = get_param(gcb,'handle');   % Get block handle
      | blk    = gcb;
      | hblock = get(h);     % Parse out handles structure
      | 
      | switch get_param(gcb,'Stype')
      |     case 'Voltage Sink'
      |         mp{3} = 'Voltage [V]';
      |     case 'Current Sink'
      |         mp{3} = 'Current [A]';
      |     case 'Angular Speed Sink'
      |         mp{3} = 'Speed [rad/s]';
      |     case 'Torque Sink'
      |         mp{3} = 'Torque [Nm]';
      |     case 'Temperature Sink'
      |         mp{3} = 'Temperature [C]';
      |     case 'Heat Flow Sink'
      |         mp{3} = 'Heat Flow [kW]';
      | end
      | set_param(gcb,'MaskPrompts',mp);
      mask Callback const:
      | en = get_param(gcb,'MaskVisibilities');
      | h      = get_param(gcb,'handle');   % Get block handle
      | blk    = gcb;
      | hblock = get(h);     % Parse out handles structure
      | 
      | switch get_param(gcb,'const')
      |     case 'on'
      |         en{3} = 'on';
      | %         delete_block([blk,'/In1'])
      | 
      |     case 'off'
      |         en{3} = 'off';
      | %         add_block('simulink/Ports & Subsystems/In1',   [blk,'/In1'],'Position',[130    -7   160     7]);         % adding inport
      | 
      | end
      | set_param(gcb,'MaskVisibilities',en);
      | 
      | % hblock.MaskPrompts{3} = 'hello';
      mask Display:
      | text(0.45,0.90,['{\bf',get_param(gcb,'Stype'),'}'],'TexMode','on','horizontalAlignment', 'center')
      | % text(0.5,0.1,['{(T)(end)}'],'TexMode','on','horizontalAlignment', 'center')
      | 
      | type = get_param(gcb,'Stype');
      | switch type
      |         case 'Voltage Sink'
      |             nm = 'Voltage [V]';
      |             id = '(V)';
      |             un = 'V';
      |         case 'Current Sink'
      |             nm = 'Current [A]';
      |             id = '(----)';
      |             un = 'A';
      |         case 'Angular Speed Sink'
      |             nm = 'Speed [rad/s]';
      |             id = '(----)';
      |             un = 'rad/s';
      |         case 'Torque Sink'
      |             nm = 'Torque [Nm]';
      |             id = '(\tau)';
      |             un = 'Nm';
      |         case 'Temperature Sink'
      |             nm = 'Temperature [C]';
      |             id = '(T)';
      |             un = 'C';
      |         case 'Heat Flow Sink'
      |             nm = 'Heat Flow [kW]';
      |             id = '(----)';
      |             un = 'kW';
      | end
      | 
      | if strcmp(get_param(gcb,'const'),'on')
      |     text(0.75,0.500,['{\bf',get_param(gcb,'Value'),un,'}'],'TexMode','on','horizontalAlignment', 'center')
      | else
      |     port_label('input',2,sprintf(['Sink ',nm]));
      | end
      | 
      | 
      | port_label('input',1,'Sink');
      | text(0.5,0.175,['{',id,' (end)}'],'TexMode','on','horizontalAlignment', 'center');
  Effort Sink12 : Subsystem  AncestorBlock=DAEMOT_Lib/Dyn Electrical Comp/Effort Sink  mask(Effort Sink (Torque)){Stype=Current Sink, const=on, value=0}
      mask prompts: Stype "Sink Type"; const "Constant Value?"; value "Current [A]"
      mask help: Used to create a effot sink.
      mask init: same as TestbedModel_v6/Effort Sink1
      settings: CopyFcn=|
      | h      = get_param(gcb,'handle');   % Get block handle
      | blk    = gcb;
      | 
      | set_param(blk, 'LinkStatus', 'inactive')
      | clear h
      | clear blk
      mask TypeOptions Stype: Voltage Sink | Current Sink | Angular Speed Sink | Torque Sink | Temperature Sink | Heat Flow Sink
      mask Callback Stype:
      | mp = get_param(gcb,'MaskPrompts');
      | h      = get_param(gcb,'handle');   % Get block handle
      | blk    = gcb;
      | hblock = get(h);     % Parse out handles structure
      | 
      | switch get_param(gcb,'Stype')
      |     case 'Voltage Sink'
      |         mp{3} = 'Voltage [V]';
      |     case 'Current Sink'
      |         mp{3} = 'Current [A]';
      |     case 'Angular Speed Sink'
      |         mp{3} = 'Speed [rad/s]';
      |     case 'Torque Sink'
      |         mp{3} = 'Torque [Nm]';
      |     case 'Temperature Sink'
      |         mp{3} = 'Temperature [C]';
      |     case 'Heat Flow Sink'
      |         mp{3} = 'Heat Flow [kW]';
      | end
      | set_param(gcb,'MaskPrompts',mp);
      mask Callback const:
      | en = get_param(gcb,'MaskVisibilities');
      | h      = get_param(gcb,'handle');   % Get block handle
      | blk    = gcb;
      | hblock = get(h);     % Parse out handles structure
      | 
      | switch get_param(gcb,'const')
      |     case 'on'
      |         en{3} = 'on';
      | %         delete_block([blk,'/In1'])
      | 
      |     case 'off'
      |         en{3} = 'off';
      | %         add_block('simulink/Ports & Subsystems/In1',   [blk,'/In1'],'Position',[130    -7   160     7]);         % adding inport
      | 
      | end
      | set_param(gcb,'MaskVisibilities',en);
      | 
      | % hblock.MaskPrompts{3} = 'hello';
      mask Display:
      | text(0.45,0.90,['{\bf',get_param(gcb,'Stype'),'}'],'TexMode','on','horizontalAlignment', 'center')
      | % text(0.5,0.1,['{(T)(end)}'],'TexMode','on','horizontalAlignment', 'center')
      | 
      | type = get_param(gcb,'Stype');
      | switch type
      |         case 'Voltage Sink'
      |             nm = 'Voltage [V]';
      |             id = '(V)';
      |             un = 'V';
      |         case 'Current Sink'
      |             nm = 'Current [A]';
      |             id = '(----)';
      |             un = 'A';
      |         case 'Angular Speed Sink'
      |             nm = 'Speed [rad/s]';
      |             id = '(----)';
      |             un = 'rad/s';
      |         case 'Torque Sink'
      |             nm = 'Torque [Nm]';
      |             id = '(\tau)';
      |             un = 'Nm';
      |         case 'Temperature Sink'
      |             nm = 'Temperature [C]';
      |             id = '(T)';
      |             un = 'C';
      |         case 'Heat Flow Sink'
      |             nm = 'Heat Flow [kW]';
      |             id = '(----)';
      |             un = 'kW';
      | end
      | 
      | if strcmp(get_param(gcb,'const'),'on')
      |     text(0.75,0.500,['{\bf',get_param(gcb,'Value'),un,'}'],'TexMode','on','horizontalAlignment', 'center')
      | else
      |     port_label('input',2,sprintf(['Sink ',nm]));
      | end
      | 
      | 
      | port_label('input',1,'Sink');
      | text(0.5,0.175,['{',id,' (end)}'],'TexMode','on','horizontalAlignment', 'center');
  Effort Sink13 : Subsystem  AncestorBlock=DAEMOT_Lib/Dyn Electrical Comp/Effort Sink  mask(Effort Sink (Torque)){Stype=Current Sink, const=off, value=0}
      mask prompts: Stype "Sink Type"; const "Constant Value?"; value "Current [A]"
      mask help: Used to create a effot sink.
      mask init: same as TestbedModel_v6/Effort Sink1
      settings: CopyFcn=|
      | h      = get_param(gcb,'handle');   % Get block handle
      | blk    = gcb;
      | 
      | set_param(blk, 'LinkStatus', 'inactive')
      | clear h
      | clear blk
      mask TypeOptions Stype: Voltage Sink | Current Sink | Angular Speed Sink | Torque Sink | Temperature Sink | Heat Flow Sink
      mask Callback Stype:
      | mp = get_param(gcb,'MaskPrompts');
      | h      = get_param(gcb,'handle');   % Get block handle
      | blk    = gcb;
      | hblock = get(h);     % Parse out handles structure
      | 
      | switch get_param(gcb,'Stype')
      |     case 'Voltage Sink'
      |         mp{3} = 'Voltage [V]';
      |     case 'Current Sink'
      |         mp{3} = 'Current [A]';
      |     case 'Angular Speed Sink'
      |         mp{3} = 'Speed [rad/s]';
      |     case 'Torque Sink'
      |         mp{3} = 'Torque [Nm]';
      |     case 'Temperature Sink'
      |         mp{3} = 'Temperature [C]';
      |     case 'Heat Flow Sink'
      |         mp{3} = 'Heat Flow [kW]';
      | end
      | set_param(gcb,'MaskPrompts',mp);
      mask Callback const:
      | en = get_param(gcb,'MaskVisibilities');
      | h      = get_param(gcb,'handle');   % Get block handle
      | blk    = gcb;
      | hblock = get(h);     % Parse out handles structure
      | 
      | switch get_param(gcb,'const')
      |     case 'on'
      |         en{3} = 'on';
      | %         delete_block([blk,'/In1'])
      | 
      |     case 'off'
      |         en{3} = 'off';
      | %         add_block('simulink/Ports & Subsystems/In1',   [blk,'/In1'],'Position',[130    -7   160     7]);         % adding inport
      | 
      | end
      | set_param(gcb,'MaskVisibilities',en);
      | 
      | % hblock.MaskPrompts{3} = 'hello';
      mask Display:
      | text(0.45,0.90,['{\bf',get_param(gcb,'Stype'),'}'],'TexMode','on','horizontalAlignment', 'center')
      | % text(0.5,0.1,['{(T)(end)}'],'TexMode','on','horizontalAlignment', 'center')
      | 
      | type = get_param(gcb,'Stype');
      | switch type
      |         case 'Voltage Sink'
      |             nm = 'Voltage [V]';
      |             id = '(V)';
      |             un = 'V';
      |         case 'Current Sink'
      |             nm = 'Current [A]';
      |             id = '(----)';
      |             un = 'A';
      |         case 'Angular Speed Sink'
      |             nm = 'Speed [rad/s]';
      |             id = '(----)';
      |             un = 'rad/s';
      |         case 'Torque Sink'
      |             nm = 'Torque [Nm]';
      |             id = '(\tau)';
      |             un = 'Nm';
      |         case 'Temperature Sink'
      |             nm = 'Temperature [C]';
      |             id = '(T)';
      |             un = 'C';
      |         case 'Heat Flow Sink'
      |             nm = 'Heat Flow [kW]';
      |             id = '(----)';
      |             un = 'kW';
      | end
      | 
      | if strcmp(get_param(gcb,'const'),'on')
      |     text(0.75,0.500,['{\bf',get_param(gcb,'Value'),un,'}'],'TexMode','on','horizontalAlignment', 'center')
      | else
      |     port_label('input',2,sprintf(['Sink ',nm]));
      | end
      | 
      | 
      | port_label('input',1,'Sink');
      | text(0.5,0.175,['{',id,' (end)}'],'TexMode','on','horizontalAlignment', 'center');
  Effort Sink14 : Subsystem  AncestorBlock=DAEMOT_Lib/Dyn Electrical Comp/Effort Sink  mask(Effort Sink (Torque)){Stype=Heat Flow Sink, const=on, value=1}
      mask prompts: Stype "Sink Type"; const "Constant Value?"; value "Heat Flow [kW]"
      mask help: Used to create a effot sink.
      mask init: same as TestbedModel_v6/Effort Sink1
      settings: CopyFcn=|
      | h      = get_param(gcb,'handle');   % Get block handle
      | blk    = gcb;
      | 
      | set_param(blk, 'LinkStatus', 'inactive')
      | clear h
      | clear blk
      mask TypeOptions Stype: Voltage Sink | Current Sink | Angular Speed Sink | Torque Sink | Temperature Sink | Heat Flow Sink
      mask Callback Stype:
      | mp = get_param(gcb,'MaskPrompts');
      | h      = get_param(gcb,'handle');   % Get block handle
      | blk    = gcb;
      | hblock = get(h);     % Parse out handles structure
      | 
      | switch get_param(gcb,'Stype')
      |     case 'Voltage Sink'
      |         mp{3} = 'Voltage [V]';
      |     case 'Current Sink'
      |         mp{3} = 'Current [A]';
      |     case 'Angular Speed Sink'
      |         mp{3} = 'Speed [rad/s]';
      |     case 'Torque Sink'
      |         mp{3} = 'Torque [Nm]';
      |     case 'Temperature Sink'
      |         mp{3} = 'Temperature [C]';
      |     case 'Heat Flow Sink'
      |         mp{3} = 'Heat Flow [kW]';
      | end
      | set_param(gcb,'MaskPrompts',mp);
      mask Callback const:
      | en = get_param(gcb,'MaskVisibilities');
      | h      = get_param(gcb,'handle');   % Get block handle
      | blk    = gcb;
      | hblock = get(h);     % Parse out handles structure
      | 
      | switch get_param(gcb,'const')
      |     case 'on'
      |         en{3} = 'on';
      | %         delete_block([blk,'/In1'])
      | 
      |     case 'off'
      |         en{3} = 'off';
      | %         add_block('simulink/Ports & Subsystems/In1',   [blk,'/In1'],'Position',[130    -7   160     7]);         % adding inport
      | 
      | end
      | set_param(gcb,'MaskVisibilities',en);
      | 
      | % hblock.MaskPrompts{3} = 'hello';
      mask Display:
      | text(0.45,0.90,['{\bf',get_param(gcb,'Stype'),'}'],'TexMode','on','horizontalAlignment', 'center')
      | % text(0.5,0.1,['{(T)(end)}'],'TexMode','on','horizontalAlignment', 'center')
      | 
      | type = get_param(gcb,'Stype');
      | switch type
      |         case 'Voltage Sink'
      |             nm = 'Voltage [V]';
      |             id = '(V)';
      |             un = 'V';
      |         case 'Current Sink'
      |             nm = 'Current [A]';
      |             id = '(----)';
      |             un = 'A';
      |         case 'Angular Speed Sink'
      |             nm = 'Speed [rad/s]';
      |             id = '(----)';
      |             un = 'rad/s';
      |         case 'Torque Sink'
      |             nm = 'Torque [Nm]';
      |             id = '(\tau)';
      |             un = 'Nm';
      |         case 'Temperature Sink'
      |             nm = 'Temperature [C]';
      |             id = '(T)';
      |             un = 'C';
      |         case 'Heat Flow Sink'
      |             nm = 'Heat Flow [kW]';
      |             id = '(----)';
      |             un = 'kW';
      | end
      | 
      | if strcmp(get_param(gcb,'const'),'on')
      |     text(0.75,0.500,['{\bf',get_param(gcb,'Value'),un,'}'],'TexMode','on','horizontalAlignment', 'center')
      | else
      |     port_label('input',2,sprintf(['Sink ',nm]));
      | end
      | 
      | 
      | port_label('input',1,'Sink');
      | text(0.5,0.175,['{',id,' (end)}'],'TexMode','on','horizontalAlignment', 'center');
  Effort Sink15 : Subsystem  AncestorBlock=DAEMOT_Lib/Dyn Electrical Comp/Effort Sink  mask(Effort Sink (Torque)){Stype=Current Sink, const=on, value=0}
      mask prompts: Stype "Sink Type"; const "Constant Value?"; value "Current [A]"
      mask help: Used to create a effot sink.
      mask init: same as TestbedModel_v6/Effort Sink1
      settings: CopyFcn=|
      | h      = get_param(gcb,'handle');   % Get block handle
      | blk    = gcb;
      | 
      | set_param(blk, 'LinkStatus', 'inactive')
      | clear h
      | clear blk
      mask TypeOptions Stype: Voltage Sink | Current Sink | Angular Speed Sink | Torque Sink | Temperature Sink | Heat Flow Sink
      mask Callback Stype:
      | mp = get_param(gcb,'MaskPrompts');
      | h      = get_param(gcb,'handle');   % Get block handle
      | blk    = gcb;
      | hblock = get(h);     % Parse out handles structure
      | 
      | switch get_param(gcb,'Stype')
      |     case 'Voltage Sink'
      |         mp{3} = 'Voltage [V]';
      |     case 'Current Sink'
      |         mp{3} = 'Current [A]';
      |     case 'Angular Speed Sink'
      |         mp{3} = 'Speed [rad/s]';
      |     case 'Torque Sink'
      |         mp{3} = 'Torque [Nm]';
      |     case 'Temperature Sink'
      |         mp{3} = 'Temperature [C]';
      |     case 'Heat Flow Sink'
      |         mp{3} = 'Heat Flow [kW]';
      | end
      | set_param(gcb,'MaskPrompts',mp);
      mask Callback const:
      | en = get_param(gcb,'MaskVisibilities');
      | h      = get_param(gcb,'handle');   % Get block handle
      | blk    = gcb;
      | hblock = get(h);     % Parse out handles structure
      | 
      | switch get_param(gcb,'const')
      |     case 'on'
      |         en{3} = 'on';
      | %         delete_block([blk,'/In1'])
      | 
      |     case 'off'
      |         en{3} = 'off';
      | %         add_block('simulink/Ports & Subsystems/In1',   [blk,'/In1'],'Position',[130    -7   160     7]);         % adding inport
      | 
      | end
      | set_param(gcb,'MaskVisibilities',en);
      | 
      | % hblock.MaskPrompts{3} = 'hello';
      mask Display:
      | text(0.45,0.90,['{\bf',get_param(gcb,'Stype'),'}'],'TexMode','on','horizontalAlignment', 'center')
      | % text(0.5,0.1,['{(T)(end)}'],'TexMode','on','horizontalAlignment', 'center')
      | 
      | type = get_param(gcb,'Stype');
      | switch type
      |         case 'Voltage Sink'
      |             nm = 'Voltage [V]';
      |             id = '(V)';
      |             un = 'V';
      |         case 'Current Sink'
      |             nm = 'Current [A]';
      |             id = '(----)';
      |             un = 'A';
      |         case 'Angular Speed Sink'
      |             nm = 'Speed [rad/s]';
      |             id = '(----)';
      |             un = 'rad/s';
      |         case 'Torque Sink'
      |             nm = 'Torque [Nm]';
      |             id = '(\tau)';
      |             un = 'Nm';
      |         case 'Temperature Sink'
      |             nm = 'Temperature [C]';
      |             id = '(T)';
      |             un = 'C';
      |         case 'Heat Flow Sink'
      |             nm = 'Heat Flow [kW]';
      |             id = '(----)';
      |             un = 'kW';
      | end
      | 
      | if strcmp(get_param(gcb,'const'),'on')
      |     text(0.75,0.500,['{\bf',get_param(gcb,'Value'),un,'}'],'TexMode','on','horizontalAlignment', 'center')
      | else
      |     port_label('input',2,sprintf(['Sink ',nm]));
      | end
      | 
      | 
      | port_label('input',1,'Sink');
      | text(0.5,0.175,['{',id,' (end)}'],'TexMode','on','horizontalAlignment', 'center');
  Effort Sink16 : Subsystem  AncestorBlock=DAEMOT_Lib/Dyn Electrical Comp/Effort Sink  mask(Effort Sink (Torque)){Stype=Angular Speed Sink, const=off, value=0}
      mask prompts: Stype "Sink Type"; const "Constant Value?"; value "Speed [rad/s]"
      mask help: Used to create a effot sink.
      mask init: same as TestbedModel_v6/Effort Sink1
      settings: CopyFcn=|
      | h      = get_param(gcb,'handle');   % Get block handle
      | blk    = gcb;
      | 
      | set_param(blk, 'LinkStatus', 'inactive')
      | clear h
      | clear blk
      mask TypeOptions Stype: Voltage Sink | Current Sink | Angular Speed Sink | Torque Sink | Temperature Sink | Heat Flow Sink
      mask Callback Stype:
      | mp = get_param(gcb,'MaskPrompts');
      | h      = get_param(gcb,'handle');   % Get block handle
      | blk    = gcb;
      | hblock = get(h);     % Parse out handles structure
      | 
      | switch get_param(gcb,'Stype')
      |     case 'Voltage Sink'
      |         mp{3} = 'Voltage [V]';
      |     case 'Current Sink'
      |         mp{3} = 'Current [A]';
      |     case 'Angular Speed Sink'
      |         mp{3} = 'Speed [rad/s]';
      |     case 'Torque Sink'
      |         mp{3} = 'Torque [Nm]';
      |     case 'Temperature Sink'
      |         mp{3} = 'Temperature [C]';
      |     case 'Heat Flow Sink'
      |         mp{3} = 'Heat Flow [kW]';
      | end
      | set_param(gcb,'MaskPrompts',mp);
      mask Callback const:
      | en = get_param(gcb,'MaskVisibilities');
      | h      = get_param(gcb,'handle');   % Get block handle
      | blk    = gcb;
      | hblock = get(h);     % Parse out handles structure
      | 
      | switch get_param(gcb,'const')
      |     case 'on'
      |         en{3} = 'on';
      | %         delete_block([blk,'/In1'])
      | 
      |     case 'off'
      |         en{3} = 'off';
      | %         add_block('simulink/Ports & Subsystems/In1',   [blk,'/In1'],'Position',[130    -7   160     7]);         % adding inport
      | 
      | end
      | set_param(gcb,'MaskVisibilities',en);
      | 
      | % hblock.MaskPrompts{3} = 'hello';
      mask Display:
      | text(0.45,0.90,['{\bf',get_param(gcb,'Stype'),'}'],'TexMode','on','horizontalAlignment', 'center')
      | % text(0.5,0.1,['{(T)(end)}'],'TexMode','on','horizontalAlignment', 'center')
      | 
      | type = get_param(gcb,'Stype');
      | switch type
      |         case 'Voltage Sink'
      |             nm = 'Voltage [V]';
      |             id = '(V)';
      |             un = 'V';
      |         case 'Current Sink'
      |             nm = 'Current [A]';
      |             id = '(----)';
      |             un = 'A';
      |         case 'Angular Speed Sink'
      |             nm = 'Speed [rad/s]';
      |             id = '(----)';
      |             un = 'rad/s';
      |         case 'Torque Sink'
      |             nm = 'Torque [Nm]';
      |             id = '(\tau)';
      |             un = 'Nm';
      |         case 'Temperature Sink'
      |             nm = 'Temperature [C]';
      |             id = '(T)';
      |             un = 'C';
      |         case 'Heat Flow Sink'
      |             nm = 'Heat Flow [kW]';
      |             id = '(----)';
      |             un = 'kW';
      | end
      | 
      | if strcmp(get_param(gcb,'const'),'on')
      |     text(0.75,0.500,['{\bf',get_param(gcb,'Value'),un,'}'],'TexMode','on','horizontalAlignment', 'center')
      | else
      |     port_label('input',2,sprintf(['Sink ',nm]));
      | end
      | 
      | 
      | port_label('input',1,'Sink');
      | text(0.5,0.175,['{',id,' (end)}'],'TexMode','on','horizontalAlignment', 'center');
  Effort Sink2 : Subsystem  AncestorBlock=DAEMOT_Lib/Dyn Electrical Comp/Effort Sink  mask(Effort Sink (Torque)){Stype=Heat Flow Sink, const=on, value=1}
      mask prompts: Stype "Sink Type"; const "Constant Value?"; value "Heat Flow [kW]"
      mask help: Used to create a effot sink.
      mask init: same as TestbedModel_v6/Effort Sink1
      settings: CopyFcn=|
      | h      = get_param(gcb,'handle');   % Get block handle
      | blk    = gcb;
      | 
      | set_param(blk, 'LinkStatus', 'inactive')
      | clear h
      | clear blk
      mask TypeOptions Stype: Voltage Sink | Current Sink | Angular Speed Sink | Torque Sink | Temperature Sink | Heat Flow Sink
      mask Callback Stype:
      | mp = get_param(gcb,'MaskPrompts');
      | h      = get_param(gcb,'handle');   % Get block handle
      | blk    = gcb;
      | hblock = get(h);     % Parse out handles structure
      | 
      | switch get_param(gcb,'Stype')
      |     case 'Voltage Sink'
      |         mp{3} = 'Voltage [V]';
      |     case 'Current Sink'
      |         mp{3} = 'Current [A]';
      |     case 'Angular Speed Sink'
      |         mp{3} = 'Speed [rad/s]';
      |     case 'Torque Sink'
      |         mp{3} = 'Torque [Nm]';
      |     case 'Temperature Sink'
      |         mp{3} = 'Temperature [C]';
      |     case 'Heat Flow Sink'
      |         mp{3} = 'Heat Flow [kW]';
      | end
      | set_param(gcb,'MaskPrompts',mp);
      mask Callback const:
      | en = get_param(gcb,'MaskVisibilities');
      | h      = get_param(gcb,'handle');   % Get block handle
      | blk    = gcb;
      | hblock = get(h);     % Parse out handles structure
      | 
      | switch get_param(gcb,'const')
      |     case 'on'
      |         en{3} = 'on';
      | %         delete_block([blk,'/In1'])
      | 
      |     case 'off'
      |         en{3} = 'off';
      | %         add_block('simulink/Ports & Subsystems/In1',   [blk,'/In1'],'Position',[130    -7   160     7]);         % adding inport
      | 
      | end
      | set_param(gcb,'MaskVisibilities',en);
      | 
      | % hblock.MaskPrompts{3} = 'hello';
      mask Display:
      | text(0.45,0.90,['{\bf',get_param(gcb,'Stype'),'}'],'TexMode','on','horizontalAlignment', 'center')
      | % text(0.5,0.1,['{(T)(end)}'],'TexMode','on','horizontalAlignment', 'center')
      | 
      | type = get_param(gcb,'Stype');
      | switch type
      |         case 'Voltage Sink'
      |             nm = 'Voltage [V]';
      |             id = '(V)';
      |             un = 'V';
      |         case 'Current Sink'
      |             nm = 'Current [A]';
      |             id = '(----)';
      |             un = 'A';
      |         case 'Angular Speed Sink'
      |             nm = 'Speed [rad/s]';
      |             id = '(----)';
      |             un = 'rad/s';
      |         case 'Torque Sink'
      |             nm = 'Torque [Nm]';
      |             id = '(\tau)';
      |             un = 'Nm';
      |         case 'Temperature Sink'
      |             nm = 'Temperature [C]';
      |             id = '(T)';
      |             un = 'C';
      |         case 'Heat Flow Sink'
      |             nm = 'Heat Flow [kW]';
      |             id = '(----)';
      |             un = 'kW';
      | end
      | 
      | if strcmp(get_param(gcb,'const'),'on')
      |     text(0.75,0.500,['{\bf',get_param(gcb,'Value'),un,'}'],'TexMode','on','horizontalAlignment', 'center')
      | else
      |     port_label('input',2,sprintf(['Sink ',nm]));
      | end
      | 
      | 
      | port_label('input',1,'Sink');
      | text(0.5,0.175,['{',id,' (end)}'],'TexMode','on','horizontalAlignment', 'center');
  Effort Sink3 : Subsystem  AncestorBlock=DAEMOT_Lib/Dyn Electrical Comp/Effort Sink  mask(Effort Sink (Torque)){Stype=Heat Flow Sink, const=on, value=1}
      mask prompts: Stype "Sink Type"; const "Constant Value?"; value "Heat Flow [kW]"
      mask help: Used to create a effot sink.
      mask init: same as TestbedModel_v6/Effort Sink1
      settings: CopyFcn=|
      | h      = get_param(gcb,'handle');   % Get block handle
      | blk    = gcb;
      | 
      | set_param(blk, 'LinkStatus', 'inactive')
      | clear h
      | clear blk
      mask TypeOptions Stype: Voltage Sink | Current Sink | Angular Speed Sink | Torque Sink | Temperature Sink | Heat Flow Sink
      mask Callback Stype:
      | mp = get_param(gcb,'MaskPrompts');
      | h      = get_param(gcb,'handle');   % Get block handle
      | blk    = gcb;
      | hblock = get(h);     % Parse out handles structure
      | 
      | switch get_param(gcb,'Stype')
      |     case 'Voltage Sink'
      |         mp{3} = 'Voltage [V]';
      |     case 'Current Sink'
      |         mp{3} = 'Current [A]';
      |     case 'Angular Speed Sink'
      |         mp{3} = 'Speed [rad/s]';
      |     case 'Torque Sink'
      |         mp{3} = 'Torque [Nm]';
      |     case 'Temperature Sink'
      |         mp{3} = 'Temperature [C]';
      |     case 'Heat Flow Sink'
      |         mp{3} = 'Heat Flow [kW]';
      | end
      | set_param(gcb,'MaskPrompts',mp);
      mask Callback const:
      | en = get_param(gcb,'MaskVisibilities');
      | h      = get_param(gcb,'handle');   % Get block handle
      | blk    = gcb;
      | hblock = get(h);     % Parse out handles structure
      | 
      | switch get_param(gcb,'const')
      |     case 'on'
      |         en{3} = 'on';
      | %         delete_block([blk,'/In1'])
      | 
      |     case 'off'
      |         en{3} = 'off';
      | %         add_block('simulink/Ports & Subsystems/In1',   [blk,'/In1'],'Position',[130    -7   160     7]);         % adding inport
      | 
      | end
      | set_param(gcb,'MaskVisibilities',en);
      | 
      | % hblock.MaskPrompts{3} = 'hello';
      mask Display:
      | text(0.45,0.90,['{\bf',get_param(gcb,'Stype'),'}'],'TexMode','on','horizontalAlignment', 'center')
      | % text(0.5,0.1,['{(T)(end)}'],'TexMode','on','horizontalAlignment', 'center')
      | 
      | type = get_param(gcb,'Stype');
      | switch type
      |         case 'Voltage Sink'
      |             nm = 'Voltage [V]';
      |             id = '(V)';
      |             un = 'V';
      |         case 'Current Sink'
      |             nm = 'Current [A]';
      |             id = '(----)';
      |             un = 'A';
      |         case 'Angular Speed Sink'
      |             nm = 'Speed [rad/s]';
      |             id = '(----)';
      |             un = 'rad/s';
      |         case 'Torque Sink'
      |             nm = 'Torque [Nm]';
      |             id = '(\tau)';
      |             un = 'Nm';
      |         case 'Temperature Sink'
      |             nm = 'Temperature [C]';
      |             id = '(T)';
      |             un = 'C';
      |         case 'Heat Flow Sink'
      |             nm = 'Heat Flow [kW]';
      |             id = '(----)';
      |             un = 'kW';
      | end
      | 
      | if strcmp(get_param(gcb,'const'),'on')
      |     text(0.75,0.500,['{\bf',get_param(gcb,'Value'),un,'}'],'TexMode','on','horizontalAlignment', 'center')
      | else
      |     port_label('input',2,sprintf(['Sink ',nm]));
      | end
      | 
      | 
      | port_label('input',1,'Sink');
      | text(0.5,0.175,['{',id,' (end)}'],'TexMode','on','horizontalAlignment', 'center');
  Effort Sink4 : Subsystem  AncestorBlock=DAEMOT_Lib/Dyn Electrical Comp/Effort Sink  mask(Effort Sink (Torque)){Stype=Voltage Sink, const=on, value=0}
      mask prompts: Stype "Sink Type"; const "Constant Value?"; value "Voltage [V]"
      mask help: Used to create a effot sink.
      mask init: same as TestbedModel_v6/Effort Sink1
      settings: CopyFcn=|
      | h      = get_param(gcb,'handle');   % Get block handle
      | blk    = gcb;
      | 
      | set_param(blk, 'LinkStatus', 'inactive')
      | clear h
      | clear blk
      mask TypeOptions Stype: Voltage Sink | Current Sink | Angular Speed Sink | Torque Sink | Temperature Sink | Heat Flow Sink
      mask Callback Stype:
      | mp = get_param(gcb,'MaskPrompts');
      | h      = get_param(gcb,'handle');   % Get block handle
      | blk    = gcb;
      | hblock = get(h);     % Parse out handles structure
      | 
      | switch get_param(gcb,'Stype')
      |     case 'Voltage Sink'
      |         mp{3} = 'Voltage [V]';
      |     case 'Current Sink'
      |         mp{3} = 'Current [A]';
      |     case 'Angular Speed Sink'
      |         mp{3} = 'Speed [rad/s]';
      |     case 'Torque Sink'
      |         mp{3} = 'Torque [Nm]';
      |     case 'Temperature Sink'
      |         mp{3} = 'Temperature [C]';
      |     case 'Heat Flow Sink'
      |         mp{3} = 'Heat Flow [kW]';
      | end
      | set_param(gcb,'MaskPrompts',mp);
      mask Callback const:
      | en = get_param(gcb,'MaskVisibilities');
      | h      = get_param(gcb,'handle');   % Get block handle
      | blk    = gcb;
      | hblock = get(h);     % Parse out handles structure
      | 
      | switch get_param(gcb,'const')
      |     case 'on'
      |         en{3} = 'on';
      | %         delete_block([blk,'/In1'])
      | 
      |     case 'off'
      |         en{3} = 'off';
      | %         add_block('simulink/Ports & Subsystems/In1',   [blk,'/In1'],'Position',[130    -7   160     7]);         % adding inport
      | 
      | end
      | set_param(gcb,'MaskVisibilities',en);
      | 
      | % hblock.MaskPrompts{3} = 'hello';
      mask Display:
      | text(0.45,0.90,['{\bf',get_param(gcb,'Stype'),'}'],'TexMode','on','horizontalAlignment', 'center')
      | % text(0.5,0.1,['{(T)(end)}'],'TexMode','on','horizontalAlignment', 'center')
      | 
      | type = get_param(gcb,'Stype');
      | switch type
      |         case 'Voltage Sink'
      |             nm = 'Voltage [V]';
      |             id = '(V)';
      |             un = 'V';
      |         case 'Current Sink'
      |             nm = 'Current [A]';
      |             id = '(----)';
      |             un = 'A';
      |         case 'Angular Speed Sink'
      |             nm = 'Speed [rad/s]';
      |             id = '(----)';
      |             un = 'rad/s';
      |         case 'Torque Sink'
      |             nm = 'Torque [Nm]';
      |             id = '(\tau)';
      |             un = 'Nm';
      |         case 'Temperature Sink'
      |             nm = 'Temperature [C]';
      |             id = '(T)';
      |             un = 'C';
      |         case 'Heat Flow Sink'
      |             nm = 'Heat Flow [kW]';
      |             id = '(----)';
      |             un = 'kW';
      | end
      | 
      | if strcmp(get_param(gcb,'const'),'on')
      |     text(0.75,0.500,['{\bf',get_param(gcb,'Value'),un,'}'],'TexMode','on','horizontalAlignment', 'center')
      | else
      |     port_label('input',2,sprintf(['Sink ',nm]));
      | end
      | 
      | 
      | port_label('input',1,'Sink');
      | text(0.5,0.175,['{',id,' (end)}'],'TexMode','on','horizontalAlignment', 'center');
  Effort Sink5 : Subsystem  AncestorBlock=DAEMOT_Lib/Dyn Electrical Comp/Effort Sink  mask(Effort Sink (Torque)){Stype=Heat Flow Sink, const=on, value=1}
      mask prompts: Stype "Sink Type"; const "Constant Value?"; value "Heat Flow [kW]"
      mask help: Used to create a effot sink.
      mask init: same as TestbedModel_v6/Effort Sink1
      settings: CopyFcn=|
      | h      = get_param(gcb,'handle');   % Get block handle
      | blk    = gcb;
      | 
      | set_param(blk, 'LinkStatus', 'inactive')
      | clear h
      | clear blk
      mask TypeOptions Stype: Voltage Sink | Current Sink | Angular Speed Sink | Torque Sink | Temperature Sink | Heat Flow Sink
      mask Callback Stype:
      | mp = get_param(gcb,'MaskPrompts');
      | h      = get_param(gcb,'handle');   % Get block handle
      | blk    = gcb;
      | hblock = get(h);     % Parse out handles structure
      | 
      | switch get_param(gcb,'Stype')
      |     case 'Voltage Sink'
      |         mp{3} = 'Voltage [V]';
      |     case 'Current Sink'
      |         mp{3} = 'Current [A]';
      |     case 'Angular Speed Sink'
      |         mp{3} = 'Speed [rad/s]';
      |     case 'Torque Sink'
      |         mp{3} = 'Torque [Nm]';
      |     case 'Temperature Sink'
      |         mp{3} = 'Temperature [C]';
      |     case 'Heat Flow Sink'
      |         mp{3} = 'Heat Flow [kW]';
      | end
      | set_param(gcb,'MaskPrompts',mp);
      mask Callback const:
      | en = get_param(gcb,'MaskVisibilities');
      | h      = get_param(gcb,'handle');   % Get block handle
      | blk    = gcb;
      | hblock = get(h);     % Parse out handles structure
      | 
      | switch get_param(gcb,'const')
      |     case 'on'
      |         en{3} = 'on';
      | %         delete_block([blk,'/In1'])
      | 
      |     case 'off'
      |         en{3} = 'off';
      | %         add_block('simulink/Ports & Subsystems/In1',   [blk,'/In1'],'Position',[130    -7   160     7]);         % adding inport
      | 
      | end
      | set_param(gcb,'MaskVisibilities',en);
      | 
      | % hblock.MaskPrompts{3} = 'hello';
      mask Display:
      | text(0.45,0.90,['{\bf',get_param(gcb,'Stype'),'}'],'TexMode','on','horizontalAlignment', 'center')
      | % text(0.5,0.1,['{(T)(end)}'],'TexMode','on','horizontalAlignment', 'center')
      | 
      | type = get_param(gcb,'Stype');
      | switch type
      |         case 'Voltage Sink'
      |             nm = 'Voltage [V]';
      |             id = '(V)';
      |             un = 'V';
      |         case 'Current Sink'
      |             nm = 'Current [A]';
      |             id = '(----)';
      |             un = 'A';
      |         case 'Angular Speed Sink'
      |             nm = 'Speed [rad/s]';
      |             id = '(----)';
      |             un = 'rad/s';
      |         case 'Torque Sink'
      |             nm = 'Torque [Nm]';
      |             id = '(\tau)';
      |             un = 'Nm';
      |         case 'Temperature Sink'
      |             nm = 'Temperature [C]';
      |             id = '(T)';
      |             un = 'C';
      |         case 'Heat Flow Sink'
      |             nm = 'Heat Flow [kW]';
      |             id = '(----)';
      |             un = 'kW';
      | end
      | 
      | if strcmp(get_param(gcb,'const'),'on')
      |     text(0.75,0.500,['{\bf',get_param(gcb,'Value'),un,'}'],'TexMode','on','horizontalAlignment', 'center')
      | else
      |     port_label('input',2,sprintf(['Sink ',nm]));
      | end
      | 
      | 
      | port_label('input',1,'Sink');
      | text(0.5,0.175,['{',id,' (end)}'],'TexMode','on','horizontalAlignment', 'center');
  Effort Sink6 : Subsystem  Commented=on  AncestorBlock=DAEMOT_Lib/Dyn Electrical Comp/Effort Sink  mask(Effort Sink (Torque)){Stype=Torque Sink, const=off, value=0}
      mask prompts: Stype "Sink Type"; const "Constant Value?"; value "Torque [Nm]"
      mask help: Used to create a effot sink.
      mask init: same as TestbedModel_v6/Effort Sink1
      settings: CopyFcn=|
      | h      = get_param(gcb,'handle');   % Get block handle
      | blk    = gcb;
      | 
      | set_param(blk, 'LinkStatus', 'inactive')
      | clear h
      | clear blk
      mask TypeOptions Stype: Voltage Sink | Current Sink | Angular Speed Sink | Torque Sink | Temperature Sink | Heat Flow Sink
      mask Callback Stype:
      | mp = get_param(gcb,'MaskPrompts');
      | h      = get_param(gcb,'handle');   % Get block handle
      | blk    = gcb;
      | hblock = get(h);     % Parse out handles structure
      | 
      | switch get_param(gcb,'Stype')
      |     case 'Voltage Sink'
      |         mp{3} = 'Voltage [V]';
      |     case 'Current Sink'
      |         mp{3} = 'Current [A]';
      |     case 'Angular Speed Sink'
      |         mp{3} = 'Speed [rad/s]';
      |     case 'Torque Sink'
      |         mp{3} = 'Torque [Nm]';
      |     case 'Temperature Sink'
      |         mp{3} = 'Temperature [C]';
      |     case 'Heat Flow Sink'
      |         mp{3} = 'Heat Flow [kW]';
      | end
      | set_param(gcb,'MaskPrompts',mp);
      mask Callback const:
      | en = get_param(gcb,'MaskVisibilities');
      | h      = get_param(gcb,'handle');   % Get block handle
      | blk    = gcb;
      | hblock = get(h);     % Parse out handles structure
      | 
      | switch get_param(gcb,'const')
      |     case 'on'
      |         en{3} = 'on';
      | %         delete_block([blk,'/In1'])
      | 
      |     case 'off'
      |         en{3} = 'off';
      | %         add_block('simulink/Ports & Subsystems/In1',   [blk,'/In1'],'Position',[130    -7   160     7]);         % adding inport
      | 
      | end
      | set_param(gcb,'MaskVisibilities',en);
      | 
      | % hblock.MaskPrompts{3} = 'hello';
      mask Display:
      | text(0.45,0.90,['{\bf',get_param(gcb,'Stype'),'}'],'TexMode','on','horizontalAlignment', 'center')
      | % text(0.5,0.1,['{(T)(end)}'],'TexMode','on','horizontalAlignment', 'center')
      | 
      | type = get_param(gcb,'Stype');
      | switch type
      |         case 'Voltage Sink'
      |             nm = 'Voltage [V]';
      |             id = '(V)';
      |             un = 'V';
      |         case 'Current Sink'
      |             nm = 'Current [A]';
      |             id = '(----)';
      |             un = 'A';
      |         case 'Angular Speed Sink'
      |             nm = 'Speed [rad/s]';
      |             id = '(----)';
      |             un = 'rad/s';
      |         case 'Torque Sink'
      |             nm = 'Torque [Nm]';
      |             id = '(\tau)';
      |             un = 'Nm';
      |         case 'Temperature Sink'
      |             nm = 'Temperature [C]';
      |             id = '(T)';
      |             un = 'C';
      |         case 'Heat Flow Sink'
      |             nm = 'Heat Flow [kW]';
      |             id = '(----)';
      |             un = 'kW';
      | end
      | 
      | if strcmp(get_param(gcb,'const'),'on')
      |     text(0.75,0.500,['{\bf',get_param(gcb,'Value'),un,'}'],'TexMode','on','horizontalAlignment', 'center')
      | else
      |     port_label('input',2,sprintf(['Sink ',nm]));
      | end
      | 
      | 
      | port_label('input',1,'Sink');
      | text(0.5,0.175,['{',id,' (end)}'],'TexMode','on','horizontalAlignment', 'center');
  Effort Sink7 : Subsystem  AncestorBlock=DAEMOT_Lib/Dyn Electrical Comp/Effort Sink  mask(Effort Sink (Torque)){Stype=Heat Flow Sink, const=on, value=1}
      mask prompts: Stype "Sink Type"; const "Constant Value?"; value "Heat Flow [kW]"
      mask help: Used to create a effot sink.
      mask init: same as TestbedModel_v6/Effort Sink1
      settings: CopyFcn=|
      | h      = get_param(gcb,'handle');   % Get block handle
      | blk    = gcb;
      | 
      | set_param(blk, 'LinkStatus', 'inactive')
      | clear h
      | clear blk
      mask TypeOptions Stype: Voltage Sink | Current Sink | Angular Speed Sink | Torque Sink | Temperature Sink | Heat Flow Sink
      mask Callback Stype:
      | mp = get_param(gcb,'MaskPrompts');
      | h      = get_param(gcb,'handle');   % Get block handle
      | blk    = gcb;
      | hblock = get(h);     % Parse out handles structure
      | 
      | switch get_param(gcb,'Stype')
      |     case 'Voltage Sink'
      |         mp{3} = 'Voltage [V]';
      |     case 'Current Sink'
      |         mp{3} = 'Current [A]';
      |     case 'Angular Speed Sink'
      |         mp{3} = 'Speed [rad/s]';
      |     case 'Torque Sink'
      |         mp{3} = 'Torque [Nm]';
      |     case 'Temperature Sink'
      |         mp{3} = 'Temperature [C]';
      |     case 'Heat Flow Sink'
      |         mp{3} = 'Heat Flow [kW]';
      | end
      | set_param(gcb,'MaskPrompts',mp);
      mask Callback const:
      | en = get_param(gcb,'MaskVisibilities');
      | h      = get_param(gcb,'handle');   % Get block handle
      | blk    = gcb;
      | hblock = get(h);     % Parse out handles structure
      | 
      | switch get_param(gcb,'const')
      |     case 'on'
      |         en{3} = 'on';
      | %         delete_block([blk,'/In1'])
      | 
      |     case 'off'
      |         en{3} = 'off';
      | %         add_block('simulink/Ports & Subsystems/In1',   [blk,'/In1'],'Position',[130    -7   160     7]);         % adding inport
      | 
      | end
      | set_param(gcb,'MaskVisibilities',en);
      | 
      | % hblock.MaskPrompts{3} = 'hello';
      mask Display:
      | text(0.45,0.90,['{\bf',get_param(gcb,'Stype'),'}'],'TexMode','on','horizontalAlignment', 'center')
      | % text(0.5,0.1,['{(T)(end)}'],'TexMode','on','horizontalAlignment', 'center')
      | 
      | type = get_param(gcb,'Stype');
      | switch type
      |         case 'Voltage Sink'
      |             nm = 'Voltage [V]';
      |             id = '(V)';
      |             un = 'V';
      |         case 'Current Sink'
      |             nm = 'Current [A]';
      |             id = '(----)';
      |             un = 'A';
      |         case 'Angular Speed Sink'
      |             nm = 'Speed [rad/s]';
      |             id = '(----)';
      |             un = 'rad/s';
      |         case 'Torque Sink'
      |             nm = 'Torque [Nm]';
      |             id = '(\tau)';
      |             un = 'Nm';
      |         case 'Temperature Sink'
      |             nm = 'Temperature [C]';
      |             id = '(T)';
      |             un = 'C';
      |         case 'Heat Flow Sink'
      |             nm = 'Heat Flow [kW]';
      |             id = '(----)';
      |             un = 'kW';
      | end
      | 
      | if strcmp(get_param(gcb,'const'),'on')
      |     text(0.75,0.500,['{\bf',get_param(gcb,'Value'),un,'}'],'TexMode','on','horizontalAlignment', 'center')
      | else
      |     port_label('input',2,sprintf(['Sink ',nm]));
      | end
      | 
      | 
      | port_label('input',1,'Sink');
      | text(0.5,0.175,['{',id,' (end)}'],'TexMode','on','horizontalAlignment', 'center');
  Effort Sink8 : Subsystem  AncestorBlock=DAEMOT_Lib/Dyn Electrical Comp/Effort Sink  mask(Effort Sink (Torque)){Stype=Heat Flow Sink, const=on, value=1}
      mask prompts: Stype "Sink Type"; const "Constant Value?"; value "Heat Flow [kW]"
      mask help: Used to create a effot sink.
      mask init: same as TestbedModel_v6/Effort Sink1
      settings: CopyFcn=|
      | h      = get_param(gcb,'handle');   % Get block handle
      | blk    = gcb;
      | 
      | set_param(blk, 'LinkStatus', 'inactive')
      | clear h
      | clear blk
      mask TypeOptions Stype: Voltage Sink | Current Sink | Angular Speed Sink | Torque Sink | Temperature Sink | Heat Flow Sink
      mask Callback Stype:
      | mp = get_param(gcb,'MaskPrompts');
      | h      = get_param(gcb,'handle');   % Get block handle
      | blk    = gcb;
      | hblock = get(h);     % Parse out handles structure
      | 
      | switch get_param(gcb,'Stype')
      |     case 'Voltage Sink'
      |         mp{3} = 'Voltage [V]';
      |     case 'Current Sink'
      |         mp{3} = 'Current [A]';
      |     case 'Angular Speed Sink'
      |         mp{3} = 'Speed [rad/s]';
      |     case 'Torque Sink'
      |         mp{3} = 'Torque [Nm]';
      |     case 'Temperature Sink'
      |         mp{3} = 'Temperature [C]';
      |     case 'Heat Flow Sink'
      |         mp{3} = 'Heat Flow [kW]';
      | end
      | set_param(gcb,'MaskPrompts',mp);
      mask Callback const:
      | en = get_param(gcb,'MaskVisibilities');
      | h      = get_param(gcb,'handle');   % Get block handle
      | blk    = gcb;
      | hblock = get(h);     % Parse out handles structure
      | 
      | switch get_param(gcb,'const')
      |     case 'on'
      |         en{3} = 'on';
      | %         delete_block([blk,'/In1'])
      | 
      |     case 'off'
      |         en{3} = 'off';
      | %         add_block('simulink/Ports & Subsystems/In1',   [blk,'/In1'],'Position',[130    -7   160     7]);         % adding inport
      | 
      | end
      | set_param(gcb,'MaskVisibilities',en);
      | 
      | % hblock.MaskPrompts{3} = 'hello';
      mask Display:
      | text(0.45,0.90,['{\bf',get_param(gcb,'Stype'),'}'],'TexMode','on','horizontalAlignment', 'center')
      | % text(0.5,0.1,['{(T)(end)}'],'TexMode','on','horizontalAlignment', 'center')
      | 
      | type = get_param(gcb,'Stype');
      | switch type
      |         case 'Voltage Sink'
      |             nm = 'Voltage [V]';
      |             id = '(V)';
      |             un = 'V';
      |         case 'Current Sink'
      |             nm = 'Current [A]';
      |             id = '(----)';
      |             un = 'A';
      |         case 'Angular Speed Sink'
      |             nm = 'Speed [rad/s]';
      |             id = '(----)';
      |             un = 'rad/s';
      |         case 'Torque Sink'
      |             nm = 'Torque [Nm]';
      |             id = '(\tau)';
      |             un = 'Nm';
      |         case 'Temperature Sink'
      |             nm = 'Temperature [C]';
      |             id = '(T)';
      |             un = 'C';
      |         case 'Heat Flow Sink'
      |             nm = 'Heat Flow [kW]';
      |             id = '(----)';
      |             un = 'kW';
      | end
      | 
      | if strcmp(get_param(gcb,'const'),'on')
      |     text(0.75,0.500,['{\bf',get_param(gcb,'Value'),un,'}'],'TexMode','on','horizontalAlignment', 'center')
      | else
      |     port_label('input',2,sprintf(['Sink ',nm]));
      | end
      | 
      | 
      | port_label('input',1,'Sink');
      | text(0.5,0.175,['{',id,' (end)}'],'TexMode','on','horizontalAlignment', 'center');
  Effort Sink9 : Subsystem  AncestorBlock=DAEMOT_Lib/Dyn Electrical Comp/Effort Sink  mask(Effort Sink (Torque)){Stype=Current Sink, const=off, value=0}
      mask prompts: Stype "Sink Type"; const "Constant Value?"; value "Current [A]"
      mask help: Used to create a effot sink.
      mask init: same as TestbedModel_v6/Effort Sink1
      settings: CopyFcn=|
      | h      = get_param(gcb,'handle');   % Get block handle
      | blk    = gcb;
      | 
      | set_param(blk, 'LinkStatus', 'inactive')
      | clear h
      | clear blk
      mask TypeOptions Stype: Voltage Sink | Current Sink | Angular Speed Sink | Torque Sink | Temperature Sink | Heat Flow Sink
      mask Callback Stype:
      | mp = get_param(gcb,'MaskPrompts');
      | h      = get_param(gcb,'handle');   % Get block handle
      | blk    = gcb;
      | hblock = get(h);     % Parse out handles structure
      | 
      | switch get_param(gcb,'Stype')
      |     case 'Voltage Sink'
      |         mp{3} = 'Voltage [V]';
      |     case 'Current Sink'
      |         mp{3} = 'Current [A]';
      |     case 'Angular Speed Sink'
      |         mp{3} = 'Speed [rad/s]';
      |     case 'Torque Sink'
      |         mp{3} = 'Torque [Nm]';
      |     case 'Temperature Sink'
      |         mp{3} = 'Temperature [C]';
      |     case 'Heat Flow Sink'
      |         mp{3} = 'Heat Flow [kW]';
      | end
      | set_param(gcb,'MaskPrompts',mp);
      mask Callback const:
      | en = get_param(gcb,'MaskVisibilities');
      | h      = get_param(gcb,'handle');   % Get block handle
      | blk    = gcb;
      | hblock = get(h);     % Parse out handles structure
      | 
      | switch get_param(gcb,'const')
      |     case 'on'
      |         en{3} = 'on';
      | %         delete_block([blk,'/In1'])
      | 
      |     case 'off'
      |         en{3} = 'off';
      | %         add_block('simulink/Ports & Subsystems/In1',   [blk,'/In1'],'Position',[130    -7   160     7]);         % adding inport
      | 
      | end
      | set_param(gcb,'MaskVisibilities',en);
      | 
      | % hblock.MaskPrompts{3} = 'hello';
      mask Display:
      | text(0.45,0.90,['{\bf',get_param(gcb,'Stype'),'}'],'TexMode','on','horizontalAlignment', 'center')
      | % text(0.5,0.1,['{(T)(end)}'],'TexMode','on','horizontalAlignment', 'center')
      | 
      | type = get_param(gcb,'Stype');
      | switch type
      |         case 'Voltage Sink'
      |             nm = 'Voltage [V]';
      |             id = '(V)';
      |             un = 'V';
      |         case 'Current Sink'
      |             nm = 'Current [A]';
      |             id = '(----)';
      |             un = 'A';
      |         case 'Angular Speed Sink'
      |             nm = 'Speed [rad/s]';
      |             id = '(----)';
      |             un = 'rad/s';
      |         case 'Torque Sink'
      |             nm = 'Torque [Nm]';
      |             id = '(\tau)';
      |             un = 'Nm';
      |         case 'Temperature Sink'
      |             nm = 'Temperature [C]';
      |             id = '(T)';
      |             un = 'C';
      |         case 'Heat Flow Sink'
      |             nm = 'Heat Flow [kW]';
      |             id = '(----)';
      |             un = 'kW';
      | end
      | 
      | if strcmp(get_param(gcb,'const'),'on')
      |     text(0.75,0.500,['{\bf',get_param(gcb,'Value'),un,'}'],'TexMode','on','horizontalAlignment', 'center')
      | else
      |     port_label('input',2,sprintf(['Sink ',nm]));
      | end
      | 
      | 
      | port_label('input',1,'Sink');
      | text(0.5,0.175,['{',id,' (end)}'],'TexMode','on','horizontalAlignment', 'center');
  Effort Source : Subsystem  AncestorBlock=DAEMOT_Lib/Dyn Electrical Comp/Effort Source  mask(Effort Source (Voltage)){Stype=Voltage Source, const=on, value=0}
      mask prompts: Stype "Source Type"; const "Constant Value?"; value "Voltage [V]"
      mask help: Used to create an effort source.
      mask init:
      | h      = get_param(gcb,'handle');   % Get block handle
      | blk    = gcb;
      | hblock = get(h);     % Parse out handles structure
      | 
      | switch Stype
      |     case 1
      |         up = 'current';
      |         dw = 'voltage';
      |     case 2
      |         dw = 'current';
      |         up = 'voltage';
      |     case 3
      |         up = 'torque';
      |         dw = 'aspeed';
      |     case 4
      |         dw = 'torque';
      |         up = 'aspeed';
      |     case 5
      |         up = 'Q_kW';
      |         dw = 'Temp';
      |     case 6
      |         dw = 'Q_kW';
      |         up = 'Temp';
      | end
      | 
      | if const == 1;
      |     try delete_block([blk,'/In1'])
      |         delete_unconnected_lines(blk);
      |         add_block('simulink/Sources/Constant',   [blk,'/val'], 'Position', [200,198,230,212]);
      |         add_line(blk,'val/1','b1/2','AutoRouting','on');
      |         set_param([blk,'/val'],'Value','value');
      | 
      |         p = get_param([blk,'/Constant'],'PortHandles');
      |         l = get_param(p.Outport,'Line');
      |         set_param(l,'Name',up);
      |         
      |         p = get_param([blk,'/val'],'PortHandles');
      |         l = get_param(p.Outport,'Line');
      |         set_param(l,'Name',dw);
      |     end
      |     p = get_param([blk,'/Constant'],'PortHandles');
      |     l = get_param(p.Outport,'Line');
      |     if strcmp(get_param(l,'name'),up)
      |     else
      |         set_param(l,'Name',up);
      |         
      |         p = get_param([blk,'/val'],'PortHandles');
      |         l = get_param(p.Outport,'Line');
      |         set_param(l,'Name',dw);
      |     end
      |      
      | %     delete_unconnected_lines(blk)
      | else
      |     try delete_block([blk,'/val'])
      |         delete_unconnected_lines(blk);
      |         add_block('simulink/Ports & Subsystems/In1',   [blk,'/In1'], 'Position', [200,198,230,212]);
      |         add_line(blk,'In1/1','b1/2','AutoRouting','on');
      |         
      |         p = get_param([blk,'/Constant'],'PortHandles');
      |         l = get_param(p.Outport,'Line');
      |         set_param(l,'Name',up);
      | 
      |         p = get_param([blk,'/In1'],'PortHandles');
      |         l = get_param(p.Outport,'Line');
      |         set_param(l,'Name',dw);
      |     end
      |     p = get_param([blk,'/Constant'],'PortHandles');
      |     l = get_param(p.Outport,'Line');
      |     if strcmp(get_param(l,'name'),up)
      |     else
      |         set_param(l,'Name',up);
      |         
      |         p = get_param([blk,'/In1'],'PortHandles');
      |         l = get_param(p.Outport,'Line');
      |         set_param(l,'Name',dw);
      |     end
      | end
      | 
      | clear h blk hblock
      settings: CopyFcn=|
      | h      = get_param(gcb,'handle');   % Get block handle
      | blk    = gcb;
      | 
      | set_param(blk, 'LinkStatus', 'inactive')
      | clear h
      | clear blk
      mask TypeOptions Stype: Voltage Source | Current Source | Angular Speed Source | Torque Source | Temperature Source | Heat Flow Source
      mask Callback Stype:
      | mp = get_param(gcb,'MaskPrompts');
      | h      = get_param(gcb,'handle');   % Get block handle
      | blk    = gcb;
      | hblock = get(h);     % Parse out handles structure
      | 
      | switch get_param(gcb,'Stype')
      |     case 'Voltage Source'
      |         mp{3} = 'Voltage [V]';
      |     case 'Current Source'
      |         mp{3} = 'Current [A]';
      |     case 'Angular Speed Source'
      |         mp{3} = 'Speed [rad/s]';
      |     case 'Torque Source'
      |         mp{3} = 'Torque [Nm]';
      |     case 'Temperature Source'
      |         mp{3} = 'Temperature [C]';
      |     case 'Heat Flow Source'
      |         mp{3} = 'Heat Flow [kW]';
      | end
      | set_param(gcb,'MaskPrompts',mp);
      mask Callback const:
      | en = get_param(gcb,'MaskVisibilities');
      | h      = get_param(gcb,'handle');   % Get block handle
      | blk    = gcb;
      | hblock = get(h);     % Parse out handles structure
      | 
      | switch get_param(gcb,'const')
      |     case 'on'
      |         en{3} = 'on';
      | %         delete_block([blk,'/In1'])
      | 
      |     case 'off'
      |         en{3} = 'off';
      | %         add_block('simulink/Ports & Subsystems/In1',   [blk,'/In1'],'Position',[130    -7   160     7]);         % adding inport
      | 
      | end
      | set_param(gcb,'MaskVisibilities',en);
      | 
      | % hblock.MaskPrompts{3} = 'hello';
      mask Display:
      | text(0.45,0.900,['{\bf',get_param(gcb,'Stype'),'}'],'TexMode','on','horizontalAlignment', 'center')
      | 
      | type = get_param(gcb,'Stype');
      | switch type
      |         case 'Voltage Source'
      |             nm = 'Voltage [V]';
      |             id = '(V)*';
      |             un = 'V';
      |         case 'Current Source'
      |             nm = 'Current [A]';
      |             id = '(----)';
      |             un = 'A';
      |         case 'Angular Speed Source'
      |             nm = 'Speed [rad/s]';
      |             id = '(----)';
      |             un = 'rad/s';
      |         case 'Torque Source'
      |             nm = 'Torque [Nm]';
      |             id = '(\tau)*';
      |             un = 'Nm';
      |         case 'Temperature Source'
      |             nm = 'Temperature [C]';
      |             id = '(T)';
      |             un = 'C';
      |         case 'Heat Flow Source'
      |             nm = 'Heat Flow [kW]';
      |             id = '(----)';
      |             un = 'kW';
      | end
      | 
      | if strcmp(get_param(gcb,'const'),'on')
      |     text(0.25,0.500,['{\bf',get_param(gcb,'Value'),un,'}'],'TexMode','on','horizontalAlignment', 'center')
      | else
      |     port_label('input',1,sprintf(['Source \n',nm]))
      | end
      | port_label('output',1,'Source')
      | text(0.5,0.175,['{(start) ',id,'}'],'TexMode','on','horizontalAlignment', 'center')
  Effort Source1 : Subsystem  AncestorBlock=DAEMOT_Lib/Dyn Electrical Comp/Effort Source  mask(Effort Source (Voltage)){Stype=Voltage Source, const=off, value=50}
      mask prompts: Stype "Source Type"; const "Constant Value?"; value "Voltage [V]"
      mask help: Used to create an effort source.
      mask init: same as TestbedModel_v6/Effort Source
      settings: CopyFcn=|
      | h      = get_param(gcb,'handle');   % Get block handle
      | blk    = gcb;
      | 
      | set_param(blk, 'LinkStatus', 'inactive')
      | clear h
      | clear blk
      mask TypeOptions Stype: Voltage Source | Current Source | Angular Speed Source | Torque Source | Temperature Source | Heat Flow Source
      mask Callback Stype:
      | mp = get_param(gcb,'MaskPrompts');
      | h      = get_param(gcb,'handle');   % Get block handle
      | blk    = gcb;
      | hblock = get(h);     % Parse out handles structure
      | 
      | switch get_param(gcb,'Stype')
      |     case 'Voltage Source'
      |         mp{3} = 'Voltage [V]';
      |     case 'Current Source'
      |         mp{3} = 'Current [A]';
      |     case 'Angular Speed Source'
      |         mp{3} = 'Speed [rad/s]';
      |     case 'Torque Source'
      |         mp{3} = 'Torque [Nm]';
      |     case 'Temperature Source'
      |         mp{3} = 'Temperature [C]';
      |     case 'Heat Flow Source'
      |         mp{3} = 'Heat Flow [kW]';
      | end
      | set_param(gcb,'MaskPrompts',mp);
      mask Callback const:
      | en = get_param(gcb,'MaskVisibilities');
      | h      = get_param(gcb,'handle');   % Get block handle
      | blk    = gcb;
      | hblock = get(h);     % Parse out handles structure
      | 
      | switch get_param(gcb,'const')
      |     case 'on'
      |         en{3} = 'on';
      | %         delete_block([blk,'/In1'])
      | 
      |     case 'off'
      |         en{3} = 'off';
      | %         add_block('simulink/Ports & Subsystems/In1',   [blk,'/In1'],'Position',[130    -7   160     7]);         % adding inport
      | 
      | end
      | set_param(gcb,'MaskVisibilities',en);
      | 
      | % hblock.MaskPrompts{3} = 'hello';
      mask Display:
      | text(0.45,0.900,['{\bf',get_param(gcb,'Stype'),'}'],'TexMode','on','horizontalAlignment', 'center')
      | 
      | type = get_param(gcb,'Stype');
      | switch type
      |         case 'Voltage Source'
      |             nm = 'Voltage [V]';
      |             id = '(V)*';
      |             un = 'V';
      |         case 'Current Source'
      |             nm = 'Current [A]';
      |             id = '(----)';
      |             un = 'A';
      |         case 'Angular Speed Source'
      |             nm = 'Speed [rad/s]';
      |             id = '(----)';
      |             un = 'rad/s';
      |         case 'Torque Source'
      |             nm = 'Torque [Nm]';
      |             id = '(\tau)*';
      |             un = 'Nm';
      |         case 'Temperature Source'
      |             nm = 'Temperature [C]';
      |             id = '(T)';
      |             un = 'C';
      |         case 'Heat Flow Source'
      |             nm = 'Heat Flow [kW]';
      |             id = '(----)';
      |             un = 'kW';
      | end
      | 
      | if strcmp(get_param(gcb,'const'),'on')
      |     text(0.25,0.500,['{\bf',get_param(gcb,'Value'),un,'}'],'TexMode','on','horizontalAlignment', 'center')
      | else
      |     port_label('input',1,sprintf(['Source \n',nm]))
      | end
      | port_label('output',1,'Source')
      | text(0.5,0.175,['{(start) ',id,'}'],'TexMode','on','horizontalAlignment', 'center')
  Gain : Gain
  Gain1 : Gain  Gain=100
  Gain10 : Gain  Gain=.05
  Gain11 : Gain  Gain=.65
  Gain12 : Gain  Commented=on  Gain=1e-2
  Gain13 : Gain  Commented=on  Gain=1e-6
  Gain2 : Gain  Gain=-1
  Gain3 : Gain
  Gain4 : Gain  Gain=100
  Gain6 : Gain  Gain=-1
  Gain7 : Gain  Gain=-1
  Gain8 : Gain
  Gain9 : Gain  Gain=100
  Goto5 : Goto  Commented=on  GotoTag=prop
  Inductor : Subsystem  AncestorBlock=DAEMOT_Lib/Dyn Electrical Comp/Inductor  mask{L=.000000001, I_initial=0}
      mask prompts: L "Inductance [H]"; I_initial "Initial Current [A]"
      mask init:
      | % if strcmp(Gn_check,'off')
      | %     %is not ground node
      | %     Gn = 0;
      | %     %V_initial = V_initial_temp;
      | % else
      | %     %is ground node
      | %     Gn = 1;
      | %     %V_initial = 0;
      | % end
      settings: CopyFcn=|
      | h      = get_param(gcb,'handle');   % Get block handle
      | blk    = gcb;
      | 
      | set_param(blk, 'LinkStatus', 'inactive')
      | clear h
      | clear blk
      mask Display:
      | image(imread('inductor.bmp'));
      | text(0.5,0.95,['{\bf Inductor}'],'TexMode','on','horizontalAlignment', 'center')
      | text(0.5,0.075,['{\bf ----}'],'TexMode','on','horizontalAlignment', 'center')
      | 
      | port_label('input',1,sprintf('Electrical \nIn'))
      | %port_label('input',2,'Inductance')
      | port_label('output',1,sprintf('Electrical \nOut'))
  Inductor1 : Subsystem  AncestorBlock=DAEMOT_Lib/Dyn Electrical Comp/Inductor  mask{L=.000000001, I_initial=5}
      mask prompts: L "Inductance [H]"; I_initial "Initial Current [A]"
      mask init:
      | % if strcmp(Gn_check,'off')
      | %     %is not ground node
      | %     Gn = 0;
      | %     %V_initial = V_initial_temp;
      | % else
      | %     %is ground node
      | %     Gn = 1;
      | %     %V_initial = 0;
      | % end
      settings: CopyFcn=|
      | h      = get_param(gcb,'handle');   % Get block handle
      | blk    = gcb;
      | 
      | set_param(blk, 'LinkStatus', 'inactive')
      | clear h
      | clear blk
      mask Display:
      | image(imread('inductor.bmp'));
      | text(0.5,0.95,['{\bf Inductor}'],'TexMode','on','horizontalAlignment', 'center')
      | text(0.5,0.075,['{\bf ----}'],'TexMode','on','horizontalAlignment', 'center')
      | 
      | port_label('input',1,sprintf('Electrical \nIn'))
      | %port_label('input',2,'Inductance')
      | port_label('output',1,sprintf('Electrical \nOut'))
  Integrator : Integrator  InitialCondition=.9
  Integrator1 : Integrator
  Integrator2 : Integrator
  Integrator3 : Integrator  InitialCondition=.5
  Integrator4 : Integrator  Commented=on
  Integrator5 : Integrator  Commented=on
  K : Gain  Commented=on  Gain=K
  Ki : Gain  Commented=on  Gain=Ki
  Kp : Gain  Commented=on  Gain=Kp
  Kv : Gain  Commented=on  Gain=1/.095
  Kv1 : Gain  Commented=on  Gain=.095
  Kv2 : Gain  Commented=on  Gain=.01
  Math Function : Math  Commented=on  Operator=magnitude^2  SaturateOnIntegerOverflow=on
  Motor : Subsystem  AncestorBlock=DAEMOT_Lib/Dyn Electrical Comp/Motor  mask{m_type=DC, R=0.019, Kv=0.095, c=0.000234, b=1.89e-05, L=1.2522e-05, I_initial=-2, Cp=60, T_initial=25}
      mask prompts: m_type "Motor Type"; R "Armature Resistance [Ohm]"; Kv "Motor Constant [Nm/A] or [V-s/rad]"; c "Static Friction Coefficient [Nm]"; b "Viscous Friction Coefficient [N*m*s/rad]"; L "Armature Inductance [H]"; I_initial "Initial Total Current [A]"; Cp "Motor Heat Capacity [J/K]"; T_initial "Initial Temperature [C]"
      mask init:
      | if m_type == 2
      |     R = R/3;
      |     L = L/3;
      | end
      settings: CopyFcn=|
      | h      = get_param(gcb,'handle');   % Get block handle
      | blk    = gcb;
      | 
      | set_param(blk, 'LinkStatus', 'inactive')
      | clear h
      | clear blk
      mask TypeOptions m_type: DC | AC
      mask Display:
      | image(imread('motor.bmp'));
      | T = get_param(gcb,'m_type');
      | if strcmp(T,'DC')
      |     text(0.5,0.95,['{\bf DC Motor}'],'TexMode','on','horizontalAlignment', 'center')
      | else
      |     text(0.5,0.95,['{\bf AC Motor}'],'TexMode','on','horizontalAlignment', 'center')
      | end
      | text(0.5,0.075,['{\bf ---- (end)}'],'TexMode','on','horizontalAlignment', 'center')
      | text(0.5,0.175,['{\bf (start) (\tau)}'],'TexMode','on','horizontalAlignment', 'center')
      | 
      | port_label('input',1,sprintf('Electrical \nIn'))
      | port_label('output',1,sprintf('Mechanical \nOut'))
      | port_label('output',2,sprintf('Cooling \nOut'))
  Motor1 : Subsystem  AncestorBlock=DAEMOT_Lib/Dyn Electrical Comp/Motor  mask{m_type=DC, R=.019, Kv=.095, c=0.000234, b=1.89e-05, L=1.2522e-05, I_initial=5, Cp=60, T_initial=25}
      mask prompts: m_type "Motor Type"; R "Armature Resistance [Ohm]"; Kv "Motor Constant [Nm/A] or [V-s/rad]"; c "Static Friction Coefficient [Nm]"; b "Viscous Friction Coefficient [N*m*s/rad]"; L "Armature Inductance [H]"; I_initial "Initial Total Current [A]"; Cp "Motor Heat Capacity [J/K]"; T_initial "Initial Temperature [C]"
      mask init:
      | if m_type == 2
      |     R = R/3;
      |     L = L/3;
      | end
      settings: CopyFcn=|
      | h      = get_param(gcb,'handle');   % Get block handle
      | blk    = gcb;
      | 
      | set_param(blk, 'LinkStatus', 'inactive')
      | clear h
      | clear blk
      mask TypeOptions m_type: DC | AC
      mask Display:
      | image(imread('motor.bmp'));
      | T = get_param(gcb,'m_type');
      | if strcmp(T,'DC')
      |     text(0.5,0.95,['{\bf DC Motor}'],'TexMode','on','horizontalAlignment', 'center')
      | else
      |     text(0.5,0.95,['{\bf AC Motor}'],'TexMode','on','horizontalAlignment', 'center')
      | end
      | text(0.5,0.075,['{\bf ---- (end)}'],'TexMode','on','horizontalAlignment', 'center')
      | text(0.5,0.175,['{\bf (start) (\tau)}'],'TexMode','on','horizontalAlignment', 'center')
      | 
      | port_label('input',1,sprintf('Electrical \nIn'))
      | port_label('output',1,sprintf('Mechanical \nOut'))
      | port_label('output',2,sprintf('Cooling \nOut'))
  Mux{,1,3..6} (6 alike) : Mux  Inputs=2
  Mux2 : Mux  Inputs=6
  Mux7 : Mux  Commented=on  Inputs=2
  Reshape : Reshape
  Reshape1 : Reshape
  Reshape2 : Reshape
  Resistor : Subsystem  AncestorBlock=DAEMOT_Lib/Dyn Electrical Comp/Resistor  mask{r_type=Voltage, Cp=60, T_initial=25}
      mask prompts: r_type "Resistor Type"; Cp "Heat Capacity [J/K]"; T_initial "Initial Temperature [C]"
      mask init:
      | h      = get_param(gcb,'handle');   % Get block handle
      | blk    = gcb;
      | hblock = get(h);     % Parse out handles structure
      | 
      | if r_type == 1
      |     set_param([blk,'/From8'],'GotoTag',char('out'));
      |     set_param([blk,'/From10'],'GotoTag',char('in'));
      |     set_param([blk,'/From12'],'GotoTag',char('out'));
      |     set_param([blk,'/From4'],'GotoTag',char('out'));
      |     set_param([blk,'/From3'],'GotoTag',char('in'));
      | else
      |     set_param([blk,'/From8'],'GotoTag',char('in'));
      |     set_param([blk,'/From10'],'GotoTag',char('out'));
      |     set_param([blk,'/From12'],'GotoTag',char('in'));
      |     set_param([blk,'/From4'],'GotoTag',char('in'));
      |     set_param([blk,'/From3'],'GotoTag',char('out'));
      | end
      settings: CopyFcn=|
      | h      = get_param(gcb,'handle');   % Get block handle
      | blk    = gcb;
      | 
      | set_param(blk, 'LinkStatus', 'inactive')
      | clear h
      | clear blk
      mask TypeOptions r_type: Voltage | Current
      mask Display:
      | image(imread('resistor.bmp'));
      | T = get_param(gcb,'r_type');
      | text(0.5,0.95,['{\bf Resistor}'],'TexMode','on','horizontalAlignment', 'center')
      | if strcmp(T,'Current')
      |     text(0.5,0.075,['{\bf (V)*}'],'TexMode','on','horizontalAlignment', 'center')
      | else
      |     text(0.5,0.075,['{\bf ----}'],'TexMode','on','horizontalAlignment', 'center')
      | end
      | port_label('input',1,sprintf('Electrical \nIn'))
      | port_label('input',2,sprintf('Resistance \n[Ohm]'))
      | port_label('output',1,sprintf('Electrical \nOut'))
      | port_label('output',2,sprintf('Cooling \nOut'))
  Saturation{,1..3} (4 alike) : Saturate  UpperLimit=.99  LowerLimit=.01
  Saturation4 : Saturate  Commented=on  UpperLimit=.99  LowerLimit=.01
  Scope{1..19,30..31,33} (22 alike) : Scope
  Scope20 : Scope  Commented=on
  Scope21 : Scope  Commented=on
  Shaft : Subsystem  AncestorBlock=DAEMOT_Lib/Dyn Electrical Comp/Shaft3  mask{J=1.09*10^-3, Num_In=1, Num_Out=1, w_initial=100, meme=off}
      mask prompts: J "Shaft Inertia"; Num_In "Number of Inputs"; Num_Out "Number of Outputs"; w_initial "Initial Speed [rad/s]"; meme "Memify"
      mask init:
      | h      = get_param(gcb,'handle');   % Get block handle
      | blk    = gcb;
      | hblock = get(h);     % Parse out handles structure
      | 
      | %%%%%%%%%%%%%%%%%%%%%%%%%%%%%% Clear Stuff %%%%%%%%%%%%%%%%%%%%%%%%%%%%%%%%
      | %delete any previous inports and bus selectors
      | for i = str2num(hblock.Num_In)+1:hblock.Ports(1)
      |     delete_block([blk,'/In',num2str(i)])
      |     delete_block([blk,'/gb',num2str(i)])
      |     delete_block([blk,'/tm',num2str(i)])
      |     delete_block([blk,'/term',num2str(i)])
      |     delete_block([blk,'/Sink',num2str(i)])
      |     delete_block([blk,'/tin',num2str(i)])
      |     
      |     delete_unconnected_lines(blk)
      | end
      | 
      | for i = str2num(hblock.Num_Out)+1:hblock.Ports(2)
      |     delete_block([blk,'/Out',num2str(i)])
      |     delete_block([blk,'/tf',num2str(i)])
      |     delete_block([blk,'/to',num2str(i)])
      |     delete_block([blk,'/b',num2str(i)])
      |     delete_block([blk,'/Source',num2str(i)])
      |     delete_block([blk,'/tg',num2str(i)])
      |     delete_block([blk,'/oo',num2str(i)])
      |     
      |     delete_unconnected_lines(blk)
      | end
      | %%%%%%%%%%%%%%%%%%%%%%%%%%%%% Clear Stuff %%%%%%%%%%%%%%%%%%%%%%%%%%%%%%%%
      | 
      | %%%%%%%%%%%%%%%%%%%%%%%%%%%%%% Edit Mux inputs %%%%%%%%%%%%%%%%%%%%%%%%%%%%%%%%
      | set_param([blk,'/Mux_In_1'],'Inputs',hblock.Num_In)
      | set_param([blk,'/Mux_In_2'],'Inputs',hblock.Num_Out)
      | % set_param([blk,'/Demux_Out_1'],'Outputs',hblock.Num_In)
      | delete_unconnected_lines(blk)
      | 
      | %%%%%%%%%%%%%%%%%%%%%%%%%%%%%% Edit Mux inputs %%%%%%%%%%%%%%%%%%%%%%%%%%%%%%%%
      | 
      | %%%%%%%%%%%%%%%%%%%%%%%%%%%%%% Create and Place Inputs %%%%%%%%%%%%%%%%%%%%%%%%%%%%%%%%
      | % generate inports, bus selectors, and route lines to each vector concat
      | for i = hblock.Ports(1)+1:str2num(hblock.Num_In)
      |     
      |     % add blocks (positioning notation [x i*s+y x+l i*s+h+y] x:(horiz. pos.), y:(vert. pos.), s:(spacing), l:(horiz. length), x:(vert. height)
      |     add_block('simulink/Ports & Subsystems/In1',   [blk,'/In',num2str(i)],    'Position',[355 i*80+425 355+30 i*80+13+425]);         % adding inport
      |     add_block([blk,'/gb1'],                        [blk,'/gb',num2str(i)],   'Position',[440 i*80+410 440+5 i*80+38+410]);         % adding inport
      |     add_block('simulink/Signal Routing/Goto',      [blk,'/tm',num2str(i)],    'Position',[500 i*80+450 500+80 i*80+14+450]);         % adding inport
      |     add_block('simulink/Sinks/Terminator',          [blk,'/term',num2str(i)],    'Position',[500 i*80+415 500+20 i*80+14+415]);         % adding inport
      |     add_block('DAEMOT_Lib/Support Functions/Sink',[blk,'/Sink',num2str(i)],'Position',[200 i*30+336 200+65 i*30+28+336]);         % adding inport
      |     add_block('simulink/Signal Routing/From',       [blk,'/tin',num2str(i)],     'Position',[-400 i*20+405 -400+80 i*20+18+405]);         % adding inport
      |     
      |     % set goto and from tags
      |     set_param([blk,'/tm',num2str(i)],'GotoTag',char(horzcat('tau_in',num2str(i))))
      |     set_param([blk,'/tin',num2str(i)],'GotoTag',char(horzcat('tau_in',num2str(i))))
      |     
      |     % set goto and from background colors
      | %    set_param([blk,'/gm',num2str(i)],'BackgroundColor','yellow')
      | %    set_param([blk,'/gt',num2str(i)],'BackgroundColor','yellow')
      | %    %set_param([blk,'/gp',num2str(i)],'BackgroundColor','yellow')
      | %    set_param([blk,'/min',num2str(i)],'BackgroundColor','yellow')
      | %    set_param([blk,'/tin',num2str(i)],'BackgroundColor','yellow')
      | %    set_param([blk,'/pout',num2str(i)],'BackgroundColor','cyan')
      |     
      |     % add lines
      |     add_line(blk,['In',num2str(i),'/1'], ['gb',num2str(i),'/1'],'AutoRouting','on')
      |     add_line(blk,['gb',num2str(i),'/2'],  ['tm',num2str(i),'/1'],'AutoRouting','on')
      |     add_line(blk,['gb',num2str(i),'/1'],  ['term',num2str(i),'/1'],'AutoRouting','on')
      |     add_line(blk,['Demux_Out_1/',num2str(1)],  ['Sink',num2str(i),'/1'],'AutoRouting','on')
      |     add_line(blk,['tin',num2str(i),'/1'],  ['Mux_In_1/',num2str(i)],'AutoRouting','on')
      |     
      | end
      | %%%%%%%%%%%%%%%%%%%%%%%%%%%%%% Create and Place Inputs %%%%%%%%%%%%%%%%%%%%%%%%%%%%%%%%
      | 
      | %%%%%%%%%%%%%%%%%%%%%%%%%%%%%% Create and Place Outputs %%%%%%%%%%%%%%%%%%%%%%%%%%%%%%%%
      | % generate inports, bus selectors, and route lines to each vector concat
      | for i = hblock.Ports(2)+1:str2num(hblock.Num_Out)
      |     
      |     % add blocks
      |     add_block('simulink/Ports & Subsystems/Out1',   [blk,'/Out',num2str(i)],   'Position',[875 i*80+425 875+30 i*80+13+425]);         % adding inport
      |     add_block('simulink/Signal Routing/Bus Creator',[blk,'/b',num2str(i)],     'Position',[825 i*80+410 825+5 i*80+38+410]);         % adding inport
      |     add_block('simulink/Signal Routing/From',       [blk,'/to',num2str(i)],     'Position',[710 i*80+435 710+80 i*80+14+435]);         % adding inport
      |     add_block('simulink/Signal Routing/From',       [blk,'/oo',num2str(i)],     'Position',[710 i*80+415 710+80 i*80+14+415]);         % adding inport
      |     add_block('simulink/Signal Routing/From',       [blk,'/tf',num2str(i)],     'Position',[935 i*20+410 935+80 i*20+18+410]);         % adding inport
      |     add_block('DAEMOT_Lib/Support Functions/Source',[blk,'/Source',num2str(i)],'Position',[1400 i*30+420 1400+65 i*30+28+420]);         % adding inport
      |     add_block('simulink/Signal Routing/Goto',       [blk,'/tg',num2str(i)],     'Position',[1550 i*30+430 1550+80 i*30+14+430]);         % adding inport
      |     
      |     % set goto and from tags
      |     set_param([blk,'/tf',num2str(i)],'GotoTag',char(horzcat('tau_out',num2str(i))))
      |     set_param([blk,'/to',num2str(i)],'GotoTag',char(horzcat('tau_out',num2str(i))))
      |     set_param([blk,'/oo',num2str(i)],'GotoTag',char(horzcat('omega')))
      |     set_param([blk,'/tg',num2str(i)],'GotoTag',char(horzcat('tau_out',num2str(i))))
      |     set_param([blk,'/b',num2str(i)],'Inputs','2')
      |     
      | %     % set goto and from background colors
      | %     set_param([blk,'/t',num2str(i)],'BackgroundColor','cyan')
      | %     set_param([blk,'/m',num2str(i)],'BackgroundColor','cyan')
      | %     set_param([blk,'/p',num2str(i)],'BackgroundColor','cyan')
      | %     set_param([blk,'/g',num2str(i)],'BackgroundColor','cyan')
      | %     set_param([blk,'/mout',num2str(i)],'BackgroundColor','cyan')
      | %     %set_param([blk,'/tout',num2str(i)],'BackgroundColor','cyan')
      | 
      |     add_line(blk,['oo',num2str(i),'/1'],['b',num2str(i),'/1'],'AutoRouting','on')
      |     p = get_param([blk,'/oo',num2str(i)],'PortHandles');
      |     l = get_param(p.Outport,'Line');
      |     set_param(l,'Name','aspeed')
      |     
      |     add_line(blk,['to',num2str(i),'/1'],['b',num2str(i),'/2'],'AutoRouting','on')
      |     p = get_param([blk,'/to',num2str(i)],'PortHandles');
      |     l = get_param(p.Outport,'Line');
      |     set_param(l,'Name','torque')
      |      
      |     add_line(blk,['b',num2str(i),'/1'],['Out',num2str(i),'/1'],'AutoRouting','on')
      |     add_line(blk,['Source',num2str(i),'/1'],['tg',num2str(i),'/1'],'AutoRouting','on')
      |     add_line(blk,['tf',num2str(i),'/1'],  ['Mux_In_2/',num2str(i)],'AutoRouting','on')
      |     
      | 
      | 
      | end
      | %%%%%%%%%%%%%%%%%%%%%%%%%%%%%% Create and Place Outputs %%%%%%%%%%%%%%%%%%%%%%%%%%%%%%%%
      | 
      | try
      |     set_param([blk,'/Selector1'],'InputPortWidth',num2str(hblock.Num_In))
      |     
      |     selector_str = '[1 ';
      |     for i = 2:str2num(hblock.Num_In)
      |         selector_str = [selector_str,num2str(i),' '];
      |     end
      |     selector_str = [selector_str,']'];
      |     set_param([blk,'/Selector1'],'IndexParamArray',{selector_str})%num2cell(1:hblock.Num_In))
      | catch
      |     selector_str = '[1 ';
      |     for i = 2:str2num(hblock.Num_In)
      |         selector_str = [selector_str,num2str(i),' '];
      |     end
      |     selector_str = [selector_str,']'];
      |     set_param([blk,'/Selector1'],'IndexParamArray',{selector_str})%num2cell(1:hblock.Num_In))
      |     
      |     set_param([blk,'/Selector1'],'InputPortWidth',num2str(hblock.Num_In))
      | end 
      |     
      | try
      |     set_param([blk,'/Selector2'],'InputPortWidth',num2str(hblock.Num_Out))
      |     
      |     selector_str = '[1 ';
      |     for i = 2:str2num(hblock.Num_Out)
      |         selector_str = [selector_str,num2str(i),' '];
      |     end
      |     selector_str = [selector_str,']'];
      |     set_param([blk,'/Selector2'],'IndexParamArray',{selector_str})%num2cell(1:hblock.Num_Out))
      | catch
      |     selector_str = '[1 ';
      |     for i = 2:str2num(hblock.Num_Out)
      |         selector_str = [selector_str,num2str(i),' '];
      |     end
      |     selector_str = [selector_str,']'];
      |     set_param([blk,'/Selector2'],'IndexParamArray',{selector_str})%num2cell(1:hblock.Num_Out))
      |     
      |     set_param([blk,'/Selector2'],'InputPortWidth',num2str(hblock.Num_Out))
      | end 
      | 
      |     clear h blk hblock
      settings: CopyFcn=|
      | h      = get_param(gcb,'handle');   % Get block handle
      | blk    = gcb;
      | 
      | set_param(blk, 'LinkStatus', 'inactive')
      | clear h
      | clear blk
      mask Display:
      | meme = get_param(gcb,'meme');
      | if strcmp(meme,'on')
      |     image(imread('ShaftMeme.bmp'));
      | else
      |     image(imread('Shaft.bmp'));
      | end
      | text(0.5,0.95,['{\bf Shaft}'],'TexMode','on','horizontalAlignment', 'center')
      | text(0.5,0.075,['{\bf ----}'],'TexMode','on','horizontalAlignment', 'center')
      | 
      | In = get_param(gcb,'Num_In');
      | Out = get_param(gcb,'Num_Out');
      | 
      | for i = 1:str2num(In)
      |     port_label('input',i,sprintf(['Mech. \nIn ',num2str(i)]))
      | end
      | 
      | for i = 1:str2num(Out)
      |     port_label('output',i,sprintf(['Mech. \nOut ',num2str(i)]))
      | end
  State Machine : Subsystem
  Step : Step  Time=.05  Before=1  After=5  SampleTime=0
  Step1 : Step  Time=10  Before=500  After=300  SampleTime=0
  Step2 : Step  Time=.375  Before=20  After=40  SampleTime=0
  Step3 : Step  Time=10  SampleTime=0
  Step4 : Step  Commented=on  Time=.25  Before=500  After=300  SampleTime=0
  Sum{,2,4..5} (4 alike) : Sum  Inputs=|+-
  Sum{1,3,6,8} (4 alike) : Sum  Inputs=|++
  Sum10 : Sum  Commented=on  Inputs=|+-
  Sum11 : Sum  Commented=on  Inputs=+++
  Sum12 : Sum  Commented=on  Inputs=|++
  Sum13 : Sum  Commented=on  Inputs=|+-
  Sum14 : Sum  Commented=on  Inputs=|++
  Sum7 : Sum  Inputs=++|
  Sum9 : Sum  Inputs=+
  Voltage Bus : Subsystem  AncestorBlock=DAEMOT_Lib/Dyn Electrical Comp/Voltage Bus  mask(Bus){Num_Out=2}
      mask prompts: Num_Out "Number of Outputs"
      mask help: This is a bus.
      mask init:
      | h      = get_param(gcb,'handle');   % Get block handle
      | blk    = gcb;
      | hblock = get(h);     % Parse out handles structure
      | 
      | %%%%%%%%%%%%%%%%%%%%%%%%%%%%%% Clear Stuff %%%%%%%%%%%%%%%%%%%%%%%%%%%%%%%%
      | % delete any previous inports and bus selectors
      | for i = str2num(hblock.Num_Out)+1:hblock.Ports(2)
      |     delete_block([blk,'/Out',num2str(i)])
      |     delete_block([blk,'/if',num2str(i)])
      |     delete_block([blk,'/io',num2str(i)])
      |     delete_block([blk,'/vo',num2str(i)])
      |     delete_block([blk,'/vot',num2str(i)])
      |     delete_block([blk,'/b',num2str(i)])
      |     delete_block([blk,'/Source',num2str(i)])
      |     delete_block([blk,'/ig',num2str(i)])
      |     delete_block([blk,'/ios',num2str(i)])
      |     delete_block([blk,'/vos',num2str(i)])
      |     
      |     delete_unconnected_lines(blk)
      | end
      | %%%%%%%%%%%%%%%%%%%%%%%%%%%%%% Clear Stuff %%%%%%%%%%%%%%%%%%%%%%%%%%%%%%%%
      | 
      | %%%%%%%%%%%%%%%%%%%%%%%%%%%%%% Edit Mux inputs %%%%%%%%%%%%%%%%%%%%%%%%%%%%%%%%
      | 
      | set_param([blk,'/Mux_In_1'],'Inputs',hblock.Num_Out)
      | set_param([blk,'/Demux_Out_1'],'Outputs',hblock.Num_Out)
      | set_param([blk,'/Bus_Sink_1'],'Inputs',num2str(str2num(hblock.Num_Out)*2))
      | 
      | %%%%%%%%%%%%%%%%%%%%%%%%%%%%%% Edit Mux inputs %%%%%%%%%%%%%%%%%%%%%%%%%%%%%%%%
      | 
      | %%%%%%%%%%%%%%%%%%%%%%%%%%%%%% Creat and Place Outputs %%%%%%%%%%%%%%%%%%%%%%%%%%%%%%%%
      | % generate inports, bus selectors, and route lines to each vector concat
      | for i = hblock.Ports(2)+1:str2num(hblock.Num_Out)
      |     
      |     % add blocks
      |     add_block('simulink/Ports & Subsystems/Out1',   [blk,'/Out',num2str(i)],   'Position',[30 i*80-25-180 60 i*80-12-180]);         % adding inport
      |     add_block('simulink/Signal Routing/From',       [blk,'/io',num2str(i)],     'Position',[-150 i*80-220 -70 i*80-202]);         % adding inport
      |     add_block('simulink/Signal Routing/From',       [blk,'/vo',num2str(i)],     'Position',[-150 i*80-20-180 -70 i*80-2-180]);         % adding inport
      |     add_block('simulink/Signal Routing/Goto',       [blk,'/vot',num2str(i)],     'Position',[1090 i*20-20-250 1170 i*20-2-250]);         % adding inport
      |     add_block('simulink/Signal Routing/From',       [blk,'/if',num2str(i)],     'Position',[25 i*20-20-400 105 i*20-2-400]);         % adding inport
      |     add_block('simulink/Signal Routing/Bus Creator',[blk,'/b',num2str(i)],     'Position',[5 i*80-20+20-218 10 i*80-2+20-198]);         % adding inport
      |     add_block('DAEMOT_Lib/Support Functions/Source',[blk,'/Source',num2str(i)],'Position',[95 i*80-214 160 i*80-186]);         % adding inport
      |     add_block('simulink/Signal Routing/Goto',       [blk,'/ig',num2str(i)],     'Position',[205 i*80-209 285 i*80-191]);         % adding inport
      |     add_block('simulink/Signal Routing/From',       [blk,'/ios',num2str(i)],     'Position',[1000 i*80-20-180 1080 i*80-2-180]);         % adding inport
      |     add_block('simulink/Signal Routing/From',       [blk,'/vos',num2str(i)],     'Position',[1000 i*80-220 1080 i*80-202]);         % adding inport
      |     
      |     % set goto and from tags
      |     set_param([blk,'/if',num2str(i)],'GotoTag',char(horzcat('I_out',num2str(i))))
      |     set_param([blk,'/io',num2str(i)],'GotoTag',char(horzcat('I_out',num2str(i))))
      |     set_param([blk,'/vo',num2str(i)],'GotoTag',char(horzcat('V_out',num2str(i))))
      |     set_param([blk,'/vot',num2str(i)],'GotoTag',char(horzcat('V_out',num2str(i))))
      |     set_param([blk,'/ig',num2str(i)],'GotoTag',char(horzcat('I_out',num2str(i))))
      |     set_param([blk,'/ios',num2str(i)],'GotoTag',char(horzcat('I_out',num2str(i))))
      |     set_param([blk,'/vos',num2str(i)],'GotoTag',char(horzcat('V_out',num2str(i))))    
      |     set_param([blk,'/b',num2str(i)],'Inputs','2')
      |     
      | %     % set goto and from background colors
      | %     set_param([blk,'/t',num2str(i)],'BackgroundColor','cyan')
      | %     set_param([blk,'/m',num2str(i)],'BackgroundColor','cyan')
      | %     set_param([blk,'/p',num2str(i)],'BackgroundColor','cyan')
      | %     set_param([blk,'/g',num2str(i)],'BackgroundColor','cyan')
      | %     set_param([blk,'/mout',num2str(i)],'BackgroundColor','cyan')
      | %     %set_param([blk,'/tout',num2str(i)],'BackgroundColor','cyan')
      |     
      |     % add lines
      |     add_line(blk,['io',num2str(i),'/1'],['b',num2str(i),'/1'],'AutoRouting','on')
      |     p = get_param([blk,'/io',num2str(i)],'PortHandles');
      |     l = get_param(p.Outport,'Line');
      |     set_param(l,'Name','current')
      |     
      |     add_line(blk,['vo',num2str(i),'/1'],['b',num2str(i),'/2'],'AutoRouting','on')
      |     p = get_param([blk,'/vo',num2str(i)],'PortHandles');
      |     l = get_param(p.Outport,'Line');
      |     set_param(l,'Name','voltage')
      |     
      |     % add lines           
      |     add_line(blk,['vos',num2str(i),'/1'],['Bus_Sink_1/',num2str(2*i-1)],'AutoRouting','on')
      |     p = get_param([blk,'/vos',num2str(i)],'PortHandles');
      |     l = get_param(p.Outport,'Line');
      |     set_param(l,'Name',['voltage',num2str(i)])
      |     
      |     add_line(blk,['ios',num2str(i),'/1'],['Bus_Sink_1/',num2str(2*i)],'AutoRouting','on')
      |     p = get_param([blk,'/ios',num2str(i)],'PortHandles');
      |     l = get_param(p.Outport,'Line');
      |     set_param(l,'Name',['current',num2str(i)])
      |      
      |     add_line(blk,['b',num2str(i),'/1'],['Out',num2str(i),'/1'],'AutoRouting','on')
      |     add_line(blk,['Source',num2str(i),'/1'],['ig',num2str(i),'/1'],'AutoRouting','on')
      |     add_line(blk,['if',num2str(i),'/1'],  ['Mux_In_1/',num2str(i)],'AutoRouting','on')
      |     add_line(blk,['Demux_Out_1/',num2str(i)],['vot',num2str(i),'/1'],'AutoRouting','on')
      |     
      | 
      | 
      | end
      | %%%%%%%%%%%%%%%%%%%%%%%%%%%%%% Create and Place Outputs %%%%%%%%%%%%%%%%%%%%%%%%%%%%%%%%
      | 
      | try
      |     set_param([blk,'/Selector1'],'InputPortWidth',num2str(hblock.Num_Out))
      |     
      |     selector_str = '[1 ';
      |     for i = 2:str2num(hblock.Num_Out)
      |         selector_str = [selector_str,num2str(i),' '];
      |     end
      |     selector_str = [selector_str,']'];
      |     set_param([blk,'/Selector1'],'IndexParamArray',{selector_str})%num2cell(1:hblock.Num_Out))
      | catch
      |     selector_str = '[1 ';
      |     for i = 2:str2num(hblock.Num_Out)
      |         selector_str = [selector_str,num2str(i),' '];
      |     end
      |     selector_str = [selector_str,']'];
      |     set_param([blk,'/Selector1'],'IndexParamArray',{selector_str})%num2cell(1:hblock.Num_Out))
      |     
      |     set_param([blk,'/Selector1'],'InputPortWidth',num2str(hblock.Num_Out))
      | end 
      |     
      |     clear h blk hblock
      settings: CopyFcn=|
      | h      = get_param(gcb,'handle');   % Get block handle
      | blk    = gcb;
      | 
      | set_param(blk, 'LinkStatus', 'inactive')
      | clear h
      | clear blk
      mask Display:
      | text(0.5,0.95,['{\bf Bus}'],'TexMode','on','horizontalAlignment', 'center')
      | text(0.5,0.075,['{\bf ----(V)}'],'TexMode','on','horizontalAlignment', 'center')
      | 
      | Out = get_param(gcb,'Num_Out');
      | 
      | port_label('input',1,sprintf(['Electrical \nIn ']))
      | port_label('input',2,'u In')
      | 
      | for i = 1:str2num(Out)
      |     port_label('output',i,sprintf(['Electrical \nOut ',num2str(i)]))
      | end
  tau : Gain  Commented=on  Gain=tau
  wires:
  Motor/2(Out2) -> Effort Sink1/1(In1)
  Converter/2(Out2) -> Effort Sink2/1(In1)
  Constant/1 -> Converter/3(In3)
  Data Manager1/1(Data) -> Scope1/1
  Data Manager2/1(Data) -> Scope2/1
  Data Manager3/1(Data) -> Scope3/1
  Converter/1(Out1) -> Motor/1(In1)
  Data Manager4/1(Data) -> Gain6/1
  Gain1/1 -> Integrator/1
  Gain/1 -> Sum1/1
  Integrator/1 -> Sum1/2
  Sum1/1 -> Saturation/1
  [dyno] -> Converter/2(In2)
  Sum/1 -> Gain1/1, Gain/1
  Data Manager5/1(Data) -> Scope5/1
  Mux/1 -> Scope6/1
  Constant1/1 -> Resistor/2(In2)
  Resistor/2(Out2) -> Effort Sink3/1(In1)
  Resistor/1(Out1) -> Effort Sink4/1(In1)
  Constant3/1 -> Converter1/3(In3)
  Converter1/2(Out2) -> Effort Sink5/1(In1)
  Gain4/1 -> Integrator1/1
  Gain3/1 -> Sum3/1
  Integrator1/1 -> Sum3/2
  Sum3/1 -> Saturation1/1
  Sum2/1 -> Gain3/1, Gain4/1
  Reshape/1 -> Bus/2(u_In)
  Constant4/1 -> Reshape/1
  Reshape1/1 -> Bus/3(u_Out)
  Converter1/1(Out1) -> Inductor/1(In1)
  Inductor/1(Out1) -> Capacitor/1(In1)
  Capacitor/1(Out1) -> Resistor/1(In1)
  [res] -> Converter1/2(In2)
  Mux1/1 -> Scope8/1
  Gain6/1 -> Mux/2, Sum/2
  Data Manager6/1(Data) -> Demux/1
  Demux/2 -> Sum2/2, Mux1/2
  Demux/1 -> Gain2/1
  Gain2/1 -> Sum2/1, Mux1/1
  Converter2/1(Out1) -> Motor1/1(In1)
  Constant6/1 -> Converter2/3(In3)
  [prop] -> Converter2/2(In2)
  Motor1/1(Out1) -> Shaft/1(In1)
  Converter2/2(Out2) -> Effort Sink8/1(In1)
  Motor1/2(Out2) -> Effort Sink7/1(In1)
  Step1/1 -> Mux6/1, Sum4/1
  Sum4/1 -> Gain11/1, Gain10/1
  Gain11/1 -> Integrator2/1
  Sum8/1 -> Saturation2/1
  Mux6/1 -> Scope30/1
  Data Manager/1(Data) -> Mux6/2, Sum4/2
  Bus/2(Out2) -> Converter2/1(In1)
  Data Manager10/1(Data) -> Scope10/1
  Data Manager9/1(Data) -> Scope11/1
  Saturation1/1 -> [res], Scope7/1
  Data Manager11/1(Data) -> Scope12/1
  Bus/6(Out6) -> Effort Sink10/1(In1)
  Bus/4(Out4) -> Effort Sink12/1(In1)
  Saturation2/1 -> [prop], Scope31/1
  Mux2/1 -> Reshape1/1
  Constant9/1 -> Mux2/6
  Constant10/1 -> Mux2/5
  Constant14/1 -> Mux2/2
  Constant15/1 -> Mux2/3
  Constant16/1 -> Mux2/4
  Saturation/1 -> [dyno], Scope4/1
  Data Manager7/1(Data) -> Scope9/1
  Data Manager8/1(Data) -> Scope13/1
  Integrator2/1 -> Sum8/2
  Gain10/1 -> Sum8/1
  Constant5/1 -> Converter3/3(In3)
  [load] -> Converter3/2(In2)
  Converter3/2(Out2) -> Effort Sink11/1(In1)
  Converter3/1(Out1) -> Inductor1/1(In1)
  Capacitor1/1(Out1) -> Effort Sink13/1(In1)
  Inductor1/1(Out1) -> Capacitor1/1(In1)
  Gain9/1 -> Integrator3/1
  Gain8/1 -> Sum6/1
  Integrator3/1 -> Sum6/2
  Sum6/1 -> Saturation3/1
  Sum5/1 -> Gain9/1, Gain8/1
  Mux3/1 -> Scope15/1
  Data Manager13/1(Data) -> Mux3/2, Sum5/2
  Constant11/1 -> Mux3/1, Sum5/1
  Saturation3/1 -> Scope14/1, [load]
  Effort Source/1(Out1) -> Battery/1(In1)
  Battery/1(Out1) -> Bus/1(In1)
  Battery/2(Out2) -> Effort Sink14/1(In1)
  Data Manager14/1(Data) -> Scope16/1
  [I_load] -> Effort Sink13/2(In2)
  Step2/1 -> [I_load]
  Bus/1(Out1) -> Effort Sink9/1(In1)
  [charge] -> Effort Sink9/2(In2)
  State Machine/1(I_lim) -> Scope17/1, Sum7/2
  State Machine/2(Switch) -> [sw]
  [sw] -> Mux2/1
  Data Manager16/1(Data) -> Mux4/1
  [bkgd] -> Effort Sink10/2(In2)
  [bkgd] -> Mux4/2
  Constant12/1 -> [bkgd]
  Mux4/1 -> State Machine/2(Bus Currents)
  Data Manager15/1(Data) -> State Machine/1(Battery)
  Sum7/1 -> Gain7/1
  Gain7/1 -> [charge]
  Data Manager18/1(Data) -> Sum7/1
  State Machine/3(state) -> Scope33/1
  Data Manager17/1(Data) -> Scope18/1
  Data Manager19/1(Data) -> Mux5/1
  [bkgd] -> Mux5/2
  Mux5/1 -> Sum9/1
  Sum9/1 -> Scope19/1
  Step4/1 -> Mux7/1, Sum10/1
  Ki/1 -> Integrator4/1
  Mux7/1 -> Scope20/1
  Data Manager20/1(Data) -> Mux7/2, Sum10/2
  Saturation4/1 -> Goto5/1, Scope21/1
  Sum10/1 -> K/1
  tau/1 -> Integrator5/1
  Integrator5/1 -> Sum12/2
  K/1 -> tau/1, Sum12/1
  Sum12/1 -> Kv/1  "tau"
  Kv/1 -> Sum13/1
  Data Manager21/1(Data) -> Sum13/2
  Sum13/1 -> Ki/1, Kp/1
  Integrator4/1 -> Sum11/3
  Kp/1 -> Sum11/2
  Data Manager22/1(Data) -> Kv1/1
  Kv1/1 -> Sum11/1
  Sum11/1 -> Kv2/1
  Kv2/1 -> Saturation4/1
  Voltage Bus/2(Out2) -> Converter1/1(In1)
  Voltage Bus/1(Out1) -> Converter/1(In1)
  Effort Source1/1(Out1) -> Voltage Bus/1(In)
  Constant17/1 -> Reshape2/1
  Reshape2/1 -> Voltage Bus/2(u)
  Data Manager23/1(Data) -> Effort Source1/1(In1)
  Bus/3(Out3) -> Converter3/1(In1)
  Bus/5(Out5) -> Effort Sink15/1(In1)
  Data Manager24/1(Data) -> Math Function/1, Gain12/1
  Math Function/1 -> Gain13/1
  Gain12/1 -> Sum14/1
  Gain13/1 -> Sum14/2
  Motor/1(Out1) -> Effort Sink16/1(In1)
  Data Manager25/1(Data) -> Effort Sink16/2(In2)
  Shaft/1(Out1) -> Air Vehicle/1(In1)
  Constant8/1 -> [AoA]
  [AoA] -> Air Vehicle/2(In2)
  Sum14/1 -> Effort Sink6/2(In2)
  Data Manager12/1(Data) -> Mux/1, Sum/1
